simulink model "Final_closeloop_sinus"  (R2024b)
settings: Solver=ode23s  StartTime=0.0  StopTime=150  RelTol=1e-3
libraries: slpidlib x16
(part 1 of 2)
settings Model: Creator=thomasmacbookpro  LastModifiedBy=thomasmacbookpro
settings OptimizationCC: ReuseModelBlockBuffer=off
settings RTWCC: GPUComputeCapability=3.5

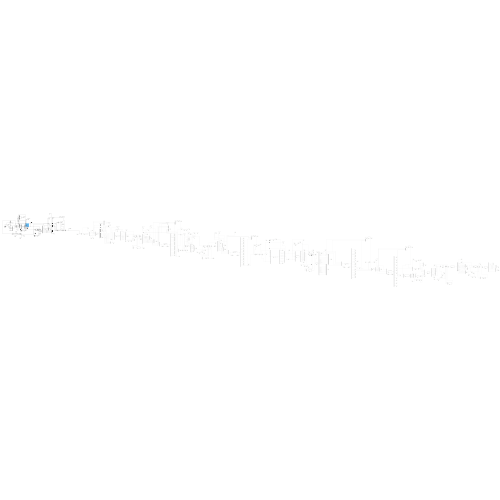
[thumbnail: Simulink's stored preview of the top-level diagram]
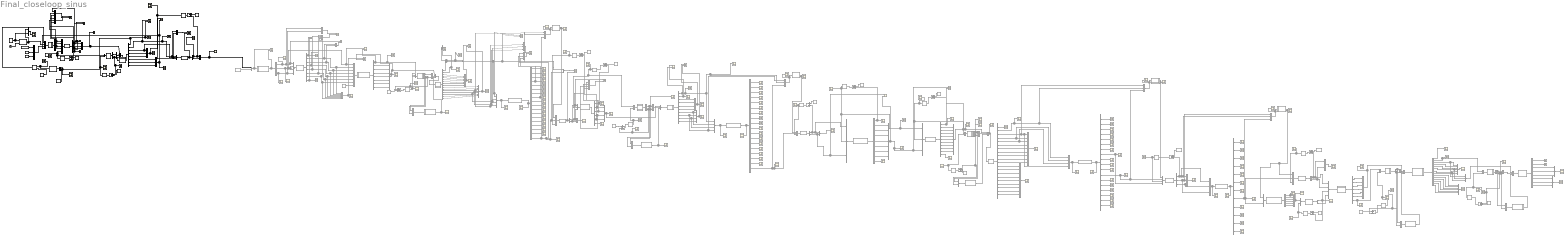
== system Final_closeloop_sinus ==
  " Q, Recycle" : Scope
  % Purge : Constant  Value=0.8
  AC-401:404 : S-Function  Commented=on  FunctionName=AC_Chromatography  Parameters=2  SFunctionDeploymentMode=off  EnableBusSupport=off
  AEX-201:204 : S-Function  Commented=on  FunctionName=AEX_Chromatography  Parameters=2  SFunctionDeploymentMode=off  EnableBusSupport=off
  AEX-301:304 : S-Function  Commented=on  FunctionName=AEX_Chromatography2  Parameters=2  SFunctionDeploymentMode=off  EnableBusSupport=off
  AEX:201:204 C : Scope  Commented=on  NumInputPorts=2
  AEX:201:204,Q IN/OUT1 : Scope  Commented=on  NumInputPorts=2
  "Area, UF-201" : Scope  Commented=on
  "Area, UF-301" : Scope  Commented=on
  "C, Glu, media [g/L]" : Constant  Value=18.1
  "C, N, media [g/L]" : Constant  Value=5.25
  "C, PE, 14" : Scope  Commented=on
  "C, PE, 22" : Scope  Commented=on
  "C, PE-1" : Scope
  "C, PE-2" : Scope  Commented=on
  "C, PE-3" : Scope  Commented=on
  "C, RE, 32" : Scope  Commented=on
  "C, RE, 4" : Scope
  "C, RE-1" : Scope  Commented=on
  "C, RE-2" : Scope  Commented=on
  "C, RE-3" : Scope  Commented=on
  "C, X, media [g/L]" : Constant  Value=0.22
  "C, alkaline lysis, out" : Scope  Commented=on
  "C, mRNA-LNP, PE, 48" : Scope  Commented=on
  "C, neutralization out" : Scope  Commented=on
  "C, output" : Scope  Commented=on
  "C,RE, 47" : Scope  Commented=on
  C,X : Scope  Commented=on
  CH3CO2K [M] : Constant  Commented=on  Value=3
  Clock : Clock
  Constant : Constant  Value=100
  Constant1 : Constant  Value=1.85
  Constant10 : Constant  Commented=on  Value=1.85
  Constant11 : Constant  Commented=on  Value=0.4507
  Constant12 : Constant  Commented=on  Value=0.2845
  Constant13 : Constant  Commented=on  Value=4.827
  Constant14 : Constant  Commented=on  Value=8
  Constant15 : Constant  Commented=on  Value=1.4
  Constant16 : Constant  Value=2.72
  Constant2 : Constant  Value=2.567
  Constant3 : Constant  Commented=on  Value=1.85
  Constant4 : Constant  Commented=on  Value=5.056
  Constant5 : Constant  Commented=on  Value=20
  Constant6 : Constant  Commented=on  Value=1.85
  Constant7 : Constant  Commented=on  Value=2.253
  Constant8 : Constant  Commented=on  Value=20
  Constant9 : Constant  Commented=on  Value=1.13
  Delay block : VariableTransportDelay  VariableDelayType=Variable transport delay  MaximumDelay=10
  Delay time : Constant  Value=0.01
  Demux : Demux  Outputs=5
  Demux1 : Demux  Outputs=8
  Demux10 : Demux  Commented=on  Outputs=18
  Demux{7,11,14,16,20,24..25,27,31} (9 alike) : Demux  Commented=on  Outputs=2
  Demux12 : Demux  Commented=on  Outputs=6
  Demux13 : Demux  Commented=on  Outputs=10
  Demux15 : Demux  Commented=on  Outputs=18
  Demux17 : Demux  Commented=on  Outputs=9
  Demux18 : Demux  Commented=on  Outputs=11
  Demux19 : Demux  Commented=on  Outputs=20
  Demux2 : Demux
  Demux21 : Demux  Commented=on  Outputs=18
  Demux22 : Demux  Commented=on  Outputs=12
  Demux23 : Demux  Commented=on  Outputs=3
  Demux26 : Demux  Commented=on  Outputs=7
  Demux28 : Demux  Commented=on  Outputs=14
  Demux29 : Demux  Commented=on  Outputs=6
  Demux3 : Demux  Outputs=2
  Demux32 : Demux  Commented=on  Outputs=8
  Demux4 : Demux  Outputs=2
  Demux5 : Demux  Commented=on  Outputs=8
  Demux6 : Demux  Commented=on  Outputs=16
  Demux8 : Demux  Commented=on  Outputs=3
  Demux9 : Demux  Commented=on  Outputs=8
  HIC-401:404 : S-Function  Commented=on  FunctionName=HIC_Chromatography  Parameters=2  SFunctionDeploymentMode=off  EnableBusSupport=off
  IVT : Scope  Commented=on
  "Input, AC-401:404" : Scope  Commented=on
  "Input, AEX-201:204" : Scope  Commented=on
  "Input, AEX-301:304" : Scope  Commented=on
  "Intput, HIC-401:404" : Scope  Commented=on
  M-101 : MATLAB Function  TreatAsAtomicUnit=on
  M-501 : S-Function  Commented=on  FunctionName=M_501  SFunctionDeploymentMode=off  EnableBusSupport=off
  MATLAB Function : MATLAB Function  Commented=on  TreatAsAtomicUnit=on
  MATLAB Function1 : MATLAB Function  Commented=on  TreatAsAtomicUnit=on
  MATLAB Function10 : MATLAB Function  Commented=on  TreatAsAtomicUnit=on
  MATLAB Function14 : MATLAB Function  Commented=on  TreatAsAtomicUnit=on
  MATLAB Function15 : MATLAB Function  Commented=on  TreatAsAtomicUnit=on
  MATLAB Function18 : MATLAB Function  Commented=on  TreatAsAtomicUnit=on
  MATLAB Function2 : MATLAB Function  Commented=on  TreatAsAtomicUnit=on
  MATLAB Function3 : MATLAB Function  Commented=on  TreatAsAtomicUnit=on
  MATLAB Function4 : MATLAB Function  Commented=on  TreatAsAtomicUnit=on
  MATLAB Function5 : MATLAB Function  Commented=on  TreatAsAtomicUnit=on
  MATLAB Function6 : MATLAB Function  Commented=on  TreatAsAtomicUnit=on
  MATLAB Function7 : MATLAB Function  Commented=on  TreatAsAtomicUnit=on
  MATLAB Function8 : MATLAB Function  TreatAsAtomicUnit=on
  MF-501 : MATLAB Function  Commented=on  TreatAsAtomicUnit=on
  MM-501 : MATLAB Function  Commented=on  TreatAsAtomicUnit=on
  Mux : Mux
  Mux{1,9..10,13..14,25,71} (7 alike) : Mux  Inputs=3
  Mux{4..6,8,11,21,79} (7 alike) : Mux  Inputs=2
  Mux{3,12,15,22,29,31..32,38,44..45,59,61..62,67..70,74..75,80..81,83,86,91} (24 alike) : Mux  Commented=on  Inputs=2
  Mux{16..17,24,41} (4 alike) : Mux  Commented=on  Inputs=7
  Mux{18,58,60,64,66} (5 alike) : Mux  Commented=on  Inputs=6
  Mux{19..20,26,30,35,39..40,42,47,49,51,56,63,72..73,76,78,84..85,87,89..90} (22 alike) : Mux  Commented=on  Inputs=3
  Mux2 : Mux  Inputs=5
  Mux23 : Mux  Commented=on  Inputs=8
  Mux{7,27,33..34,36..37,50,55,57,82,88} (11 alike) : Mux  Commented=on
  Mux43 : Mux  Commented=on  Inputs=9
  Mux46 : Mux  Commented=on  Inputs=9
  Mux48 : Mux  Commented=on  Inputs=9
  NF-501 : MATLAB Function  Commented=on  TreatAsAtomicUnit=on
  NaOH [M] : Constant  Commented=on  Value=0.42
  "Neutralization, IN/OUT2" : Scope  Commented=on  NumInputPorts=2
  Neutralization,flow IN/OUT1 : Scope  Commented=on  NumInputPorts=2
  "Output, AC-401:404" : Scope  Commented=on
  "Output, AEX-201:204" : Scope  Commented=on
  "Output, AEX-301:304" : Scope  Commented=on
  "Output, HIC-401:404" : Scope  Commented=on
  P : MATLAB Function  TreatAsAtomicUnit=on
  PID Controller : slpidlib/PID Controller  Controller=PI  Form=Parallel  TimeDomain=Continuous-time  UseExternalTs=off  SampleTime=-1  IntegratorMethod=Forward Euler  FilterMethod=Forward Euler  ControllerParametersSource=internal  P=-20  I=-30  UseKiTs=off  D=0  UseExternalDerivativeSource=off  N=100  UseFilter=on  TunerSelectOption=Transfer Function Based (PID Tuner App)  InitialConditionSource=internal  InitialConditionForIntegrator=3.33  InitialConditionForFilter=0  DifferentiatorICPrevScaledInput=0  ExternalReset=none  TrackingMode=off  Kt=1  LimitOutput=on  SatLimitsSource=internal  UpperSaturationLimit=inf  LowerSaturationLimit=-inf  LinearizeAsGain=on  AntiWindupMode=clamping  Kb=1  LimitIntegrator=off  UpperIntegratorSaturationLimit=inf  LowerIntegratorSaturationLimit=-inf  POutMin=[]  POutMax=[]  IOutMin=[]  IOutMax=[]  DOutMin=[]  DOutMax=[]  NOutMin=[]  NOutMax=[]  SumOutMin=[]  SumOutMax=[]  SaturationOutMin=[]  SaturationOutMax=[]  PParamMin=[]  PParamMax=[]  IParamMin=[]  IParamMax=[]  DParamMin=[]  DParamMax=[]  NParamMin=[]  NParamMax=[]  KbParamMin=[]  KbParamMax=[]  KtParamMin=[]  KtParamMax=[]  KbOutMin=[]  KbOutMax=[]  KtOutMin=[]  KtOutMax=[]  IntegratorOutMin=[]  IntegratorOutMax=[]  FilterOutMin=[]  FilterOutMax=[]  SumI1OutMin=[]  SumI1OutMax=[]  SumI2OutMin=[]  SumI2OutMax=[]  SumI3OutMin=[]  SumI3OutMax=[]  SumI4OutMin=[]  SumI4OutMax=[]  SumDOutMin=[]  SumDOutMax=[]  DifferentiatorOutMin=[]  DifferentiatorOutMax=[]  FilterDiffOutCoefMin=[]  FilterDiffOutCoefMax=[]  ReciprocalOutMin=[]  ReciprocalOutMax=[]  SumDenOutMin=[]  SumDenOutMax=[]  SumNumOutMin=[]  SumNumOutMax=[]  DivideOutMin=[]  DivideOutMax=[]  UdiffTsProdOutMin=[]  UdiffTsProdOutMax=[]  NTsProdOutMin=[]  NTsProdOutMax=[]  UintegralTsProdOutMin=[]  UintegralTsProdOutMax=[]  UngainTsProdOutMin=[]  UngainTsProdOutMax=[]  ClampingZeroOutDataTypeStr=Inherit: Inherit via back propagation  ClampingZeroOutMin=[]  ClampingZeroOutMax=[]  FilterDenConstantOutDataTypeStr=Inherit: Inherit via back propagation  FilterDenConstantOutMin=[]  FilterDenConstantOutMax=[]  PCopyOutDataTypeStr=Inherit: Inherit via back propagation  PCopyOutMin=[]  PCopyOutMax=[]  NCopyOutDataTypeStr=Inherit: Inherit via back propagation  NCopyOutMin=[]  NCopyOutMax=[]  IntegratorContinuousStateAttributes=''  IntegratorStateMustResolveToSignalObject=off  IntegratorRTWStateStorageClass=Auto  FilterContinuousStateAttributes=''  FilterStateMustResolveToSignalObject=off  FilterRTWStateStorageClass=Auto  ParallelPVariant=InternalParameters  IdealPVariant=Disabled  IVariant=InternalParameters  DVariant=Disabled  IntegratorVariant=Continuous  SatVariant=Enabled  AWVariant=ContClampingParallel  PCopyVariant=Disabled  TRVariant=Disabled  FdbkBlocksVariant=Forward  IdealPFdbkVariant=Disabled  SatFdbkVariant=Disabled  DerivativeFilterVariant=Disabled  NVariant=Disabled  NCopyVariant=Disabled_SignalSpec  FilterICVariant=Disabled  IntegratorICVariant=InternalICs  ExternalResetVariant=Disabled  TRSumVariant=Passthrough  SumFdbkVariant=Disabled  SumVariant=Sum_PI  TsampFilterVariant=InternalTs  TsampNgainVariant=Passthrough  TsampIntegralVariant=Disabled_SignalSpec  ExternalSaturationOutDataTypeStr=Inherit: Same as second input  DerivativeSourceVariant=Disabled  PreIntVariant=InternalPreInt
  PID Controller1 : slpidlib/PID Controller  Controller=PI  Form=Parallel  TimeDomain=Continuous-time  UseExternalTs=off  SampleTime=-1  IntegratorMethod=Forward Euler  FilterMethod=Forward Euler  ControllerParametersSource=internal  P=100  I=1762.06127367321  UseKiTs=off  D=0  UseExternalDerivativeSource=off  N=100  UseFilter=on  TunerSelectOption=Transfer Function Based (PID Tuner App)  InitialConditionSource=internal  InitialConditionForIntegrator=1134  InitialConditionForFilter=0  DifferentiatorICPrevScaledInput=0  ExternalReset=none  TrackingMode=off  Kt=1  LimitOutput=on  SatLimitsSource=internal  UpperSaturationLimit=inf  LowerSaturationLimit=-inf  LinearizeAsGain=on  AntiWindupMode=none  Kb=1  LimitIntegrator=off  UpperIntegratorSaturationLimit=inf  LowerIntegratorSaturationLimit=-inf  POutMin=[]  POutMax=[]  IOutMin=[]  IOutMax=[]  DOutMin=[]  DOutMax=[]  NOutMin=[]  NOutMax=[]  SumOutMin=[]  SumOutMax=[]  SaturationOutMin=[]  SaturationOutMax=[]  PParamMin=[]  PParamMax=[]  IParamMin=[]  IParamMax=[]  DParamMin=[]  DParamMax=[]  NParamMin=[]  NParamMax=[]  KbParamMin=[]  KbParamMax=[]  KtParamMin=[]  KtParamMax=[]  KbOutMin=[]  KbOutMax=[]  KtOutMin=[]  KtOutMax=[]  IntegratorOutMin=[]  IntegratorOutMax=[]  FilterOutMin=[]  FilterOutMax=[]  SumI1OutMin=[]  SumI1OutMax=[]  SumI2OutMin=[]  SumI2OutMax=[]  SumI3OutMin=[]  SumI3OutMax=[]  SumI4OutMin=[]  SumI4OutMax=[]  SumDOutMin=[]  SumDOutMax=[]  DifferentiatorOutMin=[]  DifferentiatorOutMax=[]  FilterDiffOutCoefMin=[]  FilterDiffOutCoefMax=[]  ReciprocalOutMin=[]  ReciprocalOutMax=[]  SumDenOutMin=[]  SumDenOutMax=[]  SumNumOutMin=[]  SumNumOutMax=[]  DivideOutMin=[]  DivideOutMax=[]  UdiffTsProdOutMin=[]  UdiffTsProdOutMax=[]  NTsProdOutMin=[]  NTsProdOutMax=[]  UintegralTsProdOutMin=[]  UintegralTsProdOutMax=[]  UngainTsProdOutMin=[]  UngainTsProdOutMax=[]  ClampingZeroOutDataTypeStr=Inherit: Inherit via back propagation  ClampingZeroOutMin=[]  ClampingZeroOutMax=[]  FilterDenConstantOutDataTypeStr=Inherit: Inherit via back propagation  FilterDenConstantOutMin=[]  FilterDenConstantOutMax=[]  PCopyOutDataTypeStr=Inherit: Inherit via back propagation  PCopyOutMin=[]  PCopyOutMax=[]  NCopyOutDataTypeStr=Inherit: Inherit via back propagation  NCopyOutMin=[]  NCopyOutMax=[]  IntegratorContinuousStateAttributes=''  IntegratorStateMustResolveToSignalObject=off  IntegratorRTWStateStorageClass=Auto  FilterContinuousStateAttributes=''  FilterStateMustResolveToSignalObject=off  FilterRTWStateStorageClass=Auto  ParallelPVariant=InternalParameters  IdealPVariant=Disabled  IVariant=InternalParameters  DVariant=Disabled  IntegratorVariant=Continuous  SatVariant=Enabled  AWVariant=Passthrough  PCopyVariant=Disabled  TRVariant=Disabled  FdbkBlocksVariant=Forward  IdealPFdbkVariant=Disabled  SatFdbkVariant=Disabled  DerivativeFilterVariant=Disabled  NVariant=Disabled  NCopyVariant=Disabled_SignalSpec  FilterICVariant=Disabled  IntegratorICVariant=InternalICs  ExternalResetVariant=Disabled  TRSumVariant=Passthrough  SumFdbkVariant=Disabled  SumVariant=Sum_PI  TsampFilterVariant=InternalTs  TsampNgainVariant=Passthrough  TsampIntegralVariant=Disabled_SignalSpec  ExternalSaturationOutDataTypeStr=Inherit: Same as second input  DerivativeSourceVariant=Disabled  PreIntVariant=InternalPreInt
  PID Controller10 : slpidlib/PID Controller  Commented=on  Controller=PI  Form=Parallel  TimeDomain=Continuous-time  UseExternalTs=off  SampleTime=-1  IntegratorMethod=Forward Euler  FilterMethod=Forward Euler  ControllerParametersSource=internal  P=0  I=1695.13781714754  UseKiTs=off  D=0  UseExternalDerivativeSource=off  N=100  UseFilter=on  TunerSelectOption=Transfer Function Based (PID Tuner App)  InitialConditionSource=internal  InitialConditionForIntegrator=1118  InitialConditionForFilter=0  DifferentiatorICPrevScaledInput=0  ExternalReset=none  TrackingMode=off  Kt=1  LimitOutput=off  SatLimitsSource=internal  UpperSaturationLimit=inf  LowerSaturationLimit=-inf  LinearizeAsGain=on  AntiWindupMode=none  Kb=1  LimitIntegrator=off  UpperIntegratorSaturationLimit=inf  LowerIntegratorSaturationLimit=-inf  POutMin=[]  POutMax=[]  IOutMin=[]  IOutMax=[]  DOutMin=[]  DOutMax=[]  NOutMin=[]  NOutMax=[]  SumOutMin=[]  SumOutMax=[]  SaturationOutMin=[]  SaturationOutMax=[]  PParamMin=[]  PParamMax=[]  IParamMin=[]  IParamMax=[]  DParamMin=[]  DParamMax=[]  NParamMin=[]  NParamMax=[]  KbParamMin=[]  KbParamMax=[]  KtParamMin=[]  KtParamMax=[]  KbOutMin=[]  KbOutMax=[]  KtOutMin=[]  KtOutMax=[]  IntegratorOutMin=[]  IntegratorOutMax=[]  FilterOutMin=[]  FilterOutMax=[]  SumI1OutMin=[]  SumI1OutMax=[]  SumI2OutMin=[]  SumI2OutMax=[]  SumI3OutMin=[]  SumI3OutMax=[]  SumI4OutMin=[]  SumI4OutMax=[]  SumDOutMin=[]  SumDOutMax=[]  DifferentiatorOutMin=[]  DifferentiatorOutMax=[]  FilterDiffOutCoefMin=[]  FilterDiffOutCoefMax=[]  ReciprocalOutMin=[]  ReciprocalOutMax=[]  SumDenOutMin=[]  SumDenOutMax=[]  SumNumOutMin=[]  SumNumOutMax=[]  DivideOutMin=[]  DivideOutMax=[]  UdiffTsProdOutMin=[]  UdiffTsProdOutMax=[]  NTsProdOutMin=[]  NTsProdOutMax=[]  UintegralTsProdOutMin=[]  UintegralTsProdOutMax=[]  UngainTsProdOutMin=[]  UngainTsProdOutMax=[]  ClampingZeroOutDataTypeStr=Inherit: Inherit via back propagation  ClampingZeroOutMin=[]  ClampingZeroOutMax=[]  FilterDenConstantOutDataTypeStr=Inherit: Inherit via back propagation  FilterDenConstantOutMin=[]  FilterDenConstantOutMax=[]  PCopyOutDataTypeStr=Inherit: Inherit via back propagation  PCopyOutMin=[]  PCopyOutMax=[]  NCopyOutDataTypeStr=Inherit: Inherit via back propagation  NCopyOutMin=[]  NCopyOutMax=[]  IntegratorContinuousStateAttributes=''  IntegratorStateMustResolveToSignalObject=off  IntegratorRTWStateStorageClass=Auto  FilterContinuousStateAttributes=''  FilterStateMustResolveToSignalObject=off  FilterRTWStateStorageClass=Auto  ParallelPVariant=InternalParameters  IdealPVariant=Disabled  IVariant=InternalParameters  DVariant=Disabled  IntegratorVariant=Continuous  SatVariant=Disabled  AWVariant=Passthrough  PCopyVariant=Disabled  TRVariant=Disabled  FdbkBlocksVariant=Forward  IdealPFdbkVariant=Disabled  SatFdbkVariant=Disabled  DerivativeFilterVariant=Disabled  NVariant=Disabled  NCopyVariant=Disabled_SignalSpec  FilterICVariant=Disabled  IntegratorICVariant=InternalICs  ExternalResetVariant=Disabled  TRSumVariant=Passthrough  SumFdbkVariant=Disabled  SumVariant=Sum_PI  TsampFilterVariant=InternalTs  TsampNgainVariant=Passthrough  TsampIntegralVariant=Disabled_SignalSpec  ExternalSaturationOutDataTypeStr=Inherit: Same as second input  DerivativeSourceVariant=Disabled  PreIntVariant=InternalPreInt
  PID Controller11 : slpidlib/PID Controller  Commented=on  Controller=PI  Form=Parallel  TimeDomain=Continuous-time  UseExternalTs=off  SampleTime=-1  IntegratorMethod=Forward Euler  FilterMethod=Forward Euler  ControllerParametersSource=internal  P=-6.6059228190806  I=-0.763863716153279  UseKiTs=off  D=0  UseExternalDerivativeSource=off  N=100  UseFilter=on  TunerSelectOption=Transfer Function Based (PID Tuner App)  InitialConditionSource=internal  InitialConditionForIntegrator=0.4507  InitialConditionForFilter=0  DifferentiatorICPrevScaledInput=0  ExternalReset=none  TrackingMode=off  Kt=1  LimitOutput=off  SatLimitsSource=internal  UpperSaturationLimit=inf  LowerSaturationLimit=-inf  LinearizeAsGain=on  AntiWindupMode=none  Kb=1  LimitIntegrator=off  UpperIntegratorSaturationLimit=inf  LowerIntegratorSaturationLimit=-inf  POutMin=[]  POutMax=[]  IOutMin=[]  IOutMax=[]  DOutMin=[]  DOutMax=[]  NOutMin=[]  NOutMax=[]  SumOutMin=[]  SumOutMax=[]  SaturationOutMin=[]  SaturationOutMax=[]  PParamMin=[]  PParamMax=[]  IParamMin=[]  IParamMax=[]  DParamMin=[]  DParamMax=[]  NParamMin=[]  NParamMax=[]  KbParamMin=[]  KbParamMax=[]  KtParamMin=[]  KtParamMax=[]  KbOutMin=[]  KbOutMax=[]  KtOutMin=[]  KtOutMax=[]  IntegratorOutMin=[]  IntegratorOutMax=[]  FilterOutMin=[]  FilterOutMax=[]  SumI1OutMin=[]  SumI1OutMax=[]  SumI2OutMin=[]  SumI2OutMax=[]  SumI3OutMin=[]  SumI3OutMax=[]  SumI4OutMin=[]  SumI4OutMax=[]  SumDOutMin=[]  SumDOutMax=[]  DifferentiatorOutMin=[]  DifferentiatorOutMax=[]  FilterDiffOutCoefMin=[]  FilterDiffOutCoefMax=[]  ReciprocalOutMin=[]  ReciprocalOutMax=[]  SumDenOutMin=[]  SumDenOutMax=[]  SumNumOutMin=[]  SumNumOutMax=[]  DivideOutMin=[]  DivideOutMax=[]  UdiffTsProdOutMin=[]  UdiffTsProdOutMax=[]  NTsProdOutMin=[]  NTsProdOutMax=[]  UintegralTsProdOutMin=[]  UintegralTsProdOutMax=[]  UngainTsProdOutMin=[]  UngainTsProdOutMax=[]  ClampingZeroOutDataTypeStr=Inherit: Inherit via back propagation  ClampingZeroOutMin=[]  ClampingZeroOutMax=[]  FilterDenConstantOutDataTypeStr=Inherit: Inherit via back propagation  FilterDenConstantOutMin=[]  FilterDenConstantOutMax=[]  PCopyOutDataTypeStr=Inherit: Inherit via back propagation  PCopyOutMin=[]  PCopyOutMax=[]  NCopyOutDataTypeStr=Inherit: Inherit via back propagation  NCopyOutMin=[]  NCopyOutMax=[]  IntegratorContinuousStateAttributes=''  IntegratorStateMustResolveToSignalObject=off  IntegratorRTWStateStorageClass=Auto  FilterContinuousStateAttributes=''  FilterStateMustResolveToSignalObject=off  FilterRTWStateStorageClass=Auto  ParallelPVariant=InternalParameters  IdealPVariant=Disabled  IVariant=InternalParameters  DVariant=Disabled  IntegratorVariant=Continuous  SatVariant=Disabled  AWVariant=Passthrough  PCopyVariant=Disabled  TRVariant=Disabled  FdbkBlocksVariant=Forward  IdealPFdbkVariant=Disabled  SatFdbkVariant=Disabled  DerivativeFilterVariant=Disabled  NVariant=Disabled  NCopyVariant=Disabled_SignalSpec  FilterICVariant=Disabled  IntegratorICVariant=InternalICs  ExternalResetVariant=Disabled  TRSumVariant=Passthrough  SumFdbkVariant=Disabled  SumVariant=Sum_PI  TsampFilterVariant=InternalTs  TsampNgainVariant=Passthrough  TsampIntegralVariant=Disabled_SignalSpec  ExternalSaturationOutDataTypeStr=Inherit: Same as second input  DerivativeSourceVariant=Disabled  PreIntVariant=InternalPreInt
  PID Controller12 : slpidlib/PID Controller  Commented=on  Controller=PI  Form=Parallel  TimeDomain=Continuous-time  UseExternalTs=off  SampleTime=-1  IntegratorMethod=Forward Euler  FilterMethod=Forward Euler  ControllerParametersSource=internal  P=-6.9172503700087  I=-0.837559909578323  UseKiTs=off  D=0  UseExternalDerivativeSource=off  N=100  UseFilter=on  TunerSelectOption=Transfer Function Based (PID Tuner App)  InitialConditionSource=internal  InitialConditionForIntegrator=0.2845  InitialConditionForFilter=0  DifferentiatorICPrevScaledInput=0  ExternalReset=none  TrackingMode=off  Kt=1  LimitOutput=off  SatLimitsSource=internal  UpperSaturationLimit=inf  LowerSaturationLimit=-inf  LinearizeAsGain=on  AntiWindupMode=none  Kb=1  LimitIntegrator=off  UpperIntegratorSaturationLimit=inf  LowerIntegratorSaturationLimit=-inf  POutMin=[]  POutMax=[]  IOutMin=[]  IOutMax=[]  DOutMin=[]  DOutMax=[]  NOutMin=[]  NOutMax=[]  SumOutMin=[]  SumOutMax=[]  SaturationOutMin=[]  SaturationOutMax=[]  PParamMin=[]  PParamMax=[]  IParamMin=[]  IParamMax=[]  DParamMin=[]  DParamMax=[]  NParamMin=[]  NParamMax=[]  KbParamMin=[]  KbParamMax=[]  KtParamMin=[]  KtParamMax=[]  KbOutMin=[]  KbOutMax=[]  KtOutMin=[]  KtOutMax=[]  IntegratorOutMin=[]  IntegratorOutMax=[]  FilterOutMin=[]  FilterOutMax=[]  SumI1OutMin=[]  SumI1OutMax=[]  SumI2OutMin=[]  SumI2OutMax=[]  SumI3OutMin=[]  SumI3OutMax=[]  SumI4OutMin=[]  SumI4OutMax=[]  SumDOutMin=[]  SumDOutMax=[]  DifferentiatorOutMin=[]  DifferentiatorOutMax=[]  FilterDiffOutCoefMin=[]  FilterDiffOutCoefMax=[]  ReciprocalOutMin=[]  ReciprocalOutMax=[]  SumDenOutMin=[]  SumDenOutMax=[]  SumNumOutMin=[]  SumNumOutMax=[]  DivideOutMin=[]  DivideOutMax=[]  UdiffTsProdOutMin=[]  UdiffTsProdOutMax=[]  NTsProdOutMin=[]  NTsProdOutMax=[]  UintegralTsProdOutMin=[]  UintegralTsProdOutMax=[]  UngainTsProdOutMin=[]  UngainTsProdOutMax=[]  ClampingZeroOutDataTypeStr=Inherit: Inherit via back propagation  ClampingZeroOutMin=[]  ClampingZeroOutMax=[]  FilterDenConstantOutDataTypeStr=Inherit: Inherit via back propagation  FilterDenConstantOutMin=[]  FilterDenConstantOutMax=[]  PCopyOutDataTypeStr=Inherit: Inherit via back propagation  PCopyOutMin=[]  PCopyOutMax=[]  NCopyOutDataTypeStr=Inherit: Inherit via back propagation  NCopyOutMin=[]  NCopyOutMax=[]  IntegratorContinuousStateAttributes=''  IntegratorStateMustResolveToSignalObject=off  IntegratorRTWStateStorageClass=Auto  FilterContinuousStateAttributes=''  FilterStateMustResolveToSignalObject=off  FilterRTWStateStorageClass=Auto  ParallelPVariant=InternalParameters  IdealPVariant=Disabled  IVariant=InternalParameters  DVariant=Disabled  IntegratorVariant=Continuous  SatVariant=Disabled  AWVariant=Passthrough  PCopyVariant=Disabled  TRVariant=Disabled  FdbkBlocksVariant=Forward  IdealPFdbkVariant=Disabled  SatFdbkVariant=Disabled  DerivativeFilterVariant=Disabled  NVariant=Disabled  NCopyVariant=Disabled_SignalSpec  FilterICVariant=Disabled  IntegratorICVariant=InternalICs  ExternalResetVariant=Disabled  TRSumVariant=Passthrough  SumFdbkVariant=Disabled  SumVariant=Sum_PI  TsampFilterVariant=InternalTs  TsampNgainVariant=Passthrough  TsampIntegralVariant=Disabled_SignalSpec  ExternalSaturationOutDataTypeStr=Inherit: Same as second input  DerivativeSourceVariant=Disabled  PreIntVariant=InternalPreInt
  PID Controller13 : slpidlib/PID Controller  Commented=on  Controller=PI  Form=Parallel  TimeDomain=Continuous-time  UseExternalTs=off  SampleTime=-1  IntegratorMethod=Forward Euler  FilterMethod=Forward Euler  ControllerParametersSource=internal  P=-6.91725036983727  I=-0.837559909557566  UseKiTs=off  D=0  UseExternalDerivativeSource=off  N=100  UseFilter=on  TunerSelectOption=Transfer Function Based (PID Tuner App)  InitialConditionSource=internal  InitialConditionForIntegrator=4  InitialConditionForFilter=0  DifferentiatorICPrevScaledInput=0  ExternalReset=none  TrackingMode=off  Kt=1  LimitOutput=off  SatLimitsSource=internal  UpperSaturationLimit=inf  LowerSaturationLimit=-inf  LinearizeAsGain=on  AntiWindupMode=none  Kb=1  LimitIntegrator=off  UpperIntegratorSaturationLimit=inf  LowerIntegratorSaturationLimit=-inf  POutMin=[]  POutMax=[]  IOutMin=[]  IOutMax=[]  DOutMin=[]  DOutMax=[]  NOutMin=[]  NOutMax=[]  SumOutMin=[]  SumOutMax=[]  SaturationOutMin=[]  SaturationOutMax=[]  PParamMin=[]  PParamMax=[]  IParamMin=[]  IParamMax=[]  DParamMin=[]  DParamMax=[]  NParamMin=[]  NParamMax=[]  KbParamMin=[]  KbParamMax=[]  KtParamMin=[]  KtParamMax=[]  KbOutMin=[]  KbOutMax=[]  KtOutMin=[]  KtOutMax=[]  IntegratorOutMin=[]  IntegratorOutMax=[]  FilterOutMin=[]  FilterOutMax=[]  SumI1OutMin=[]  SumI1OutMax=[]  SumI2OutMin=[]  SumI2OutMax=[]  SumI3OutMin=[]  SumI3OutMax=[]  SumI4OutMin=[]  SumI4OutMax=[]  SumDOutMin=[]  SumDOutMax=[]  DifferentiatorOutMin=[]  DifferentiatorOutMax=[]  FilterDiffOutCoefMin=[]  FilterDiffOutCoefMax=[]  ReciprocalOutMin=[]  ReciprocalOutMax=[]  SumDenOutMin=[]  SumDenOutMax=[]  SumNumOutMin=[]  SumNumOutMax=[]  DivideOutMin=[]  DivideOutMax=[]  UdiffTsProdOutMin=[]  UdiffTsProdOutMax=[]  NTsProdOutMin=[]  NTsProdOutMax=[]  UintegralTsProdOutMin=[]  UintegralTsProdOutMax=[]  UngainTsProdOutMin=[]  UngainTsProdOutMax=[]  ClampingZeroOutDataTypeStr=Inherit: Inherit via back propagation  ClampingZeroOutMin=[]  ClampingZeroOutMax=[]  FilterDenConstantOutDataTypeStr=Inherit: Inherit via back propagation  FilterDenConstantOutMin=[]  FilterDenConstantOutMax=[]  PCopyOutDataTypeStr=Inherit: Inherit via back propagation  PCopyOutMin=[]  PCopyOutMax=[]  NCopyOutDataTypeStr=Inherit: Inherit via back propagation  NCopyOutMin=[]  NCopyOutMax=[]  IntegratorContinuousStateAttributes=''  IntegratorStateMustResolveToSignalObject=off  IntegratorRTWStateStorageClass=Auto  FilterContinuousStateAttributes=''  FilterStateMustResolveToSignalObject=off  FilterRTWStateStorageClass=Auto  ParallelPVariant=InternalParameters  IdealPVariant=Disabled  IVariant=InternalParameters  DVariant=Disabled  IntegratorVariant=Continuous  SatVariant=Disabled  AWVariant=Passthrough  PCopyVariant=Disabled  TRVariant=Disabled  FdbkBlocksVariant=Forward  IdealPFdbkVariant=Disabled  SatFdbkVariant=Disabled  DerivativeFilterVariant=Disabled  NVariant=Disabled  NCopyVariant=Disabled_SignalSpec  FilterICVariant=Disabled  IntegratorICVariant=InternalICs  ExternalResetVariant=Disabled  TRSumVariant=Passthrough  SumFdbkVariant=Disabled  SumVariant=Sum_PI  TsampFilterVariant=InternalTs  TsampNgainVariant=Passthrough  TsampIntegralVariant=Disabled_SignalSpec  ExternalSaturationOutDataTypeStr=Inherit: Same as second input  DerivativeSourceVariant=Disabled  PreIntVariant=InternalPreInt
  PID Controller14 : slpidlib/PID Controller  Commented=on  Controller=PI  Form=Parallel  TimeDomain=Continuous-time  UseExternalTs=off  SampleTime=-1  IntegratorMethod=Forward Euler  FilterMethod=Forward Euler  ControllerParametersSource=internal  P=0  I=1138.66901210131  UseKiTs=off  D=0  UseExternalDerivativeSource=off  N=100  UseFilter=on  TunerSelectOption=Transfer Function Based (PID Tuner App)  InitialConditionSource=internal  InitialConditionForIntegrator=2334  InitialConditionForFilter=0  DifferentiatorICPrevScaledInput=0  ExternalReset=none  TrackingMode=off  Kt=1  LimitOutput=off  SatLimitsSource=internal  UpperSaturationLimit=inf  LowerSaturationLimit=-inf  LinearizeAsGain=on  AntiWindupMode=none  Kb=1  LimitIntegrator=off  UpperIntegratorSaturationLimit=inf  LowerIntegratorSaturationLimit=-inf  POutMin=[]  POutMax=[]  IOutMin=[]  IOutMax=[]  DOutMin=[]  DOutMax=[]  NOutMin=[]  NOutMax=[]  SumOutMin=[]  SumOutMax=[]  SaturationOutMin=[]  SaturationOutMax=[]  PParamMin=[]  PParamMax=[]  IParamMin=[]  IParamMax=[]  DParamMin=[]  DParamMax=[]  NParamMin=[]  NParamMax=[]  KbParamMin=[]  KbParamMax=[]  KtParamMin=[]  KtParamMax=[]  KbOutMin=[]  KbOutMax=[]  KtOutMin=[]  KtOutMax=[]  IntegratorOutMin=[]  IntegratorOutMax=[]  FilterOutMin=[]  FilterOutMax=[]  SumI1OutMin=[]  SumI1OutMax=[]  SumI2OutMin=[]  SumI2OutMax=[]  SumI3OutMin=[]  SumI3OutMax=[]  SumI4OutMin=[]  SumI4OutMax=[]  SumDOutMin=[]  SumDOutMax=[]  DifferentiatorOutMin=[]  DifferentiatorOutMax=[]  FilterDiffOutCoefMin=[]  FilterDiffOutCoefMax=[]  ReciprocalOutMin=[]  ReciprocalOutMax=[]  SumDenOutMin=[]  SumDenOutMax=[]  SumNumOutMin=[]  SumNumOutMax=[]  DivideOutMin=[]  DivideOutMax=[]  UdiffTsProdOutMin=[]  UdiffTsProdOutMax=[]  NTsProdOutMin=[]  NTsProdOutMax=[]  UintegralTsProdOutMin=[]  UintegralTsProdOutMax=[]  UngainTsProdOutMin=[]  UngainTsProdOutMax=[]  ClampingZeroOutDataTypeStr=Inherit: Inherit via back propagation  ClampingZeroOutMin=[]  ClampingZeroOutMax=[]  FilterDenConstantOutDataTypeStr=Inherit: Inherit via back propagation  FilterDenConstantOutMin=[]  FilterDenConstantOutMax=[]  PCopyOutDataTypeStr=Inherit: Inherit via back propagation  PCopyOutMin=[]  PCopyOutMax=[]  NCopyOutDataTypeStr=Inherit: Inherit via back propagation  NCopyOutMin=[]  NCopyOutMax=[]  IntegratorContinuousStateAttributes=''  IntegratorStateMustResolveToSignalObject=off  IntegratorRTWStateStorageClass=Auto  FilterContinuousStateAttributes=''  FilterStateMustResolveToSignalObject=off  FilterRTWStateStorageClass=Auto  ParallelPVariant=InternalParameters  IdealPVariant=Disabled  IVariant=InternalParameters  DVariant=Disabled  IntegratorVariant=Continuous  SatVariant=Disabled  AWVariant=Passthrough  PCopyVariant=Disabled  TRVariant=Disabled  FdbkBlocksVariant=Forward  IdealPFdbkVariant=Disabled  SatFdbkVariant=Disabled  DerivativeFilterVariant=Disabled  NVariant=Disabled  NCopyVariant=Disabled_SignalSpec  FilterICVariant=Disabled  IntegratorICVariant=InternalICs  ExternalResetVariant=Disabled  TRSumVariant=Passthrough  SumFdbkVariant=Disabled  SumVariant=Sum_PI  TsampFilterVariant=InternalTs  TsampNgainVariant=Passthrough  TsampIntegralVariant=Disabled_SignalSpec  ExternalSaturationOutDataTypeStr=Inherit: Same as second input  DerivativeSourceVariant=Disabled  PreIntVariant=InternalPreInt
  PID Controller15 : slpidlib/PID Controller  Commented=on  Controller=PI  Form=Parallel  TimeDomain=Continuous-time  UseExternalTs=off  SampleTime=-1  IntegratorMethod=Forward Euler  FilterMethod=Forward Euler  ControllerParametersSource=internal  P=0  I=2710.16235928108  UseKiTs=off  D=0  UseExternalDerivativeSource=off  N=100  UseFilter=on  TunerSelectOption=Transfer Function Based (PID Tuner App)  InitialConditionSource=internal  InitialConditionForIntegrator=964.3  InitialConditionForFilter=0  DifferentiatorICPrevScaledInput=0  ExternalReset=none  TrackingMode=off  Kt=1  LimitOutput=off  SatLimitsSource=internal  UpperSaturationLimit=inf  LowerSaturationLimit=-inf  LinearizeAsGain=on  AntiWindupMode=none  Kb=1  LimitIntegrator=off  UpperIntegratorSaturationLimit=inf  LowerIntegratorSaturationLimit=-inf  POutMin=[]  POutMax=[]  IOutMin=[]  IOutMax=[]  DOutMin=[]  DOutMax=[]  NOutMin=[]  NOutMax=[]  SumOutMin=[]  SumOutMax=[]  SaturationOutMin=[]  SaturationOutMax=[]  PParamMin=[]  PParamMax=[]  IParamMin=[]  IParamMax=[]  DParamMin=[]  DParamMax=[]  NParamMin=[]  NParamMax=[]  KbParamMin=[]  KbParamMax=[]  KtParamMin=[]  KtParamMax=[]  KbOutMin=[]  KbOutMax=[]  KtOutMin=[]  KtOutMax=[]  IntegratorOutMin=[]  IntegratorOutMax=[]  FilterOutMin=[]  FilterOutMax=[]  SumI1OutMin=[]  SumI1OutMax=[]  SumI2OutMin=[]  SumI2OutMax=[]  SumI3OutMin=[]  SumI3OutMax=[]  SumI4OutMin=[]  SumI4OutMax=[]  SumDOutMin=[]  SumDOutMax=[]  DifferentiatorOutMin=[]  DifferentiatorOutMax=[]  FilterDiffOutCoefMin=[]  FilterDiffOutCoefMax=[]  ReciprocalOutMin=[]  ReciprocalOutMax=[]  SumDenOutMin=[]  SumDenOutMax=[]  SumNumOutMin=[]  SumNumOutMax=[]  DivideOutMin=[]  DivideOutMax=[]  UdiffTsProdOutMin=[]  UdiffTsProdOutMax=[]  NTsProdOutMin=[]  NTsProdOutMax=[]  UintegralTsProdOutMin=[]  UintegralTsProdOutMax=[]  UngainTsProdOutMin=[]  UngainTsProdOutMax=[]  ClampingZeroOutDataTypeStr=Inherit: Inherit via back propagation  ClampingZeroOutMin=[]  ClampingZeroOutMax=[]  FilterDenConstantOutDataTypeStr=Inherit: Inherit via back propagation  FilterDenConstantOutMin=[]  FilterDenConstantOutMax=[]  PCopyOutDataTypeStr=Inherit: Inherit via back propagation  PCopyOutMin=[]  PCopyOutMax=[]  NCopyOutDataTypeStr=Inherit: Inherit via back propagation  NCopyOutMin=[]  NCopyOutMax=[]  IntegratorContinuousStateAttributes=''  IntegratorStateMustResolveToSignalObject=off  IntegratorRTWStateStorageClass=Auto  FilterContinuousStateAttributes=''  FilterStateMustResolveToSignalObject=off  FilterRTWStateStorageClass=Auto  ParallelPVariant=InternalParameters  IdealPVariant=Disabled  IVariant=InternalParameters  DVariant=Disabled  IntegratorVariant=Continuous  SatVariant=Disabled  AWVariant=Passthrough  PCopyVariant=Disabled  TRVariant=Disabled  FdbkBlocksVariant=Forward  IdealPFdbkVariant=Disabled  SatFdbkVariant=Disabled  DerivativeFilterVariant=Disabled  NVariant=Disabled  NCopyVariant=Disabled_SignalSpec  FilterICVariant=Disabled  IntegratorICVariant=InternalICs  ExternalResetVariant=Disabled  TRSumVariant=Passthrough  SumFdbkVariant=Disabled  SumVariant=Sum_PI  TsampFilterVariant=InternalTs  TsampNgainVariant=Passthrough  TsampIntegralVariant=Disabled_SignalSpec  ExternalSaturationOutDataTypeStr=Inherit: Same as second input  DerivativeSourceVariant=Disabled  PreIntVariant=InternalPreInt
  PID Controller2 : slpidlib/PID Controller  Controller=PI  Form=Parallel  TimeDomain=Continuous-time  UseExternalTs=off  SampleTime=-1  IntegratorMethod=Forward Euler  FilterMethod=Forward Euler  ControllerParametersSource=internal  P=-7.18723566147925  I=-6.57758159914682  UseKiTs=off  D=0  UseExternalDerivativeSource=off  N=100  UseFilter=on  TunerSelectOption=Transfer Function Based (PID Tuner App)  InitialConditionSource=internal  InitialConditionForIntegrator=0  InitialConditionForFilter=0  DifferentiatorICPrevScaledInput=0  ExternalReset=none  TrackingMode=off  Kt=1  LimitOutput=off  SatLimitsSource=internal  UpperSaturationLimit=inf  LowerSaturationLimit=-inf  LinearizeAsGain=on  AntiWindupMode=none  Kb=1  LimitIntegrator=off  UpperIntegratorSaturationLimit=inf  LowerIntegratorSaturationLimit=-inf  POutMin=[]  POutMax=[]  IOutMin=[]  IOutMax=[]  DOutMin=[]  DOutMax=[]  NOutMin=[]  NOutMax=[]  SumOutMin=[]  SumOutMax=[]  SaturationOutMin=[]  SaturationOutMax=[]  PParamMin=[]  PParamMax=[]  IParamMin=[]  IParamMax=[]  DParamMin=[]  DParamMax=[]  NParamMin=[]  NParamMax=[]  KbParamMin=[]  KbParamMax=[]  KtParamMin=[]  KtParamMax=[]  KbOutMin=[]  KbOutMax=[]  KtOutMin=[]  KtOutMax=[]  IntegratorOutMin=[]  IntegratorOutMax=[]  FilterOutMin=[]  FilterOutMax=[]  SumI1OutMin=[]  SumI1OutMax=[]  SumI2OutMin=[]  SumI2OutMax=[]  SumI3OutMin=[]  SumI3OutMax=[]  SumI4OutMin=[]  SumI4OutMax=[]  SumDOutMin=[]  SumDOutMax=[]  DifferentiatorOutMin=[]  DifferentiatorOutMax=[]  FilterDiffOutCoefMin=[]  FilterDiffOutCoefMax=[]  ReciprocalOutMin=[]  ReciprocalOutMax=[]  SumDenOutMin=[]  SumDenOutMax=[]  SumNumOutMin=[]  SumNumOutMax=[]  DivideOutMin=[]  DivideOutMax=[]  UdiffTsProdOutMin=[]  UdiffTsProdOutMax=[]  NTsProdOutMin=[]  NTsProdOutMax=[]  UintegralTsProdOutMin=[]  UintegralTsProdOutMax=[]  UngainTsProdOutMin=[]  UngainTsProdOutMax=[]  ClampingZeroOutDataTypeStr=Inherit: Inherit via back propagation  ClampingZeroOutMin=[]  ClampingZeroOutMax=[]  FilterDenConstantOutDataTypeStr=Inherit: Inherit via back propagation  FilterDenConstantOutMin=[]  FilterDenConstantOutMax=[]  PCopyOutDataTypeStr=Inherit: Inherit via back propagation  PCopyOutMin=[]  PCopyOutMax=[]  NCopyOutDataTypeStr=Inherit: Inherit via back propagation  NCopyOutMin=[]  NCopyOutMax=[]  IntegratorContinuousStateAttributes=''  IntegratorStateMustResolveToSignalObject=off  IntegratorRTWStateStorageClass=Auto  FilterContinuousStateAttributes=''  FilterStateMustResolveToSignalObject=off  FilterRTWStateStorageClass=Auto  ParallelPVariant=InternalParameters  IdealPVariant=Disabled  IVariant=InternalParameters  DVariant=Disabled  IntegratorVariant=Continuous  SatVariant=Disabled  AWVariant=Passthrough  PCopyVariant=Disabled  TRVariant=Disabled  FdbkBlocksVariant=Forward  IdealPFdbkVariant=Disabled  SatFdbkVariant=Disabled  DerivativeFilterVariant=Disabled  NVariant=Disabled  NCopyVariant=Disabled_SignalSpec  FilterICVariant=Disabled  IntegratorICVariant=InternalICs  ExternalResetVariant=Disabled  TRSumVariant=Passthrough  SumFdbkVariant=Disabled  SumVariant=Sum_PI  TsampFilterVariant=InternalTs  TsampNgainVariant=Passthrough  TsampIntegralVariant=Disabled_SignalSpec  ExternalSaturationOutDataTypeStr=Inherit: Same as second input  DerivativeSourceVariant=Disabled  PreIntVariant=InternalPreInt
  PID Controller3 : slpidlib/PID Controller  Commented=on  Controller=PI  Form=Parallel  TimeDomain=Continuous-time  UseExternalTs=off  SampleTime=-1  IntegratorMethod=Forward Euler  FilterMethod=Forward Euler  ControllerParametersSource=internal  P=0  I=238.210092745493  UseKiTs=off  D=0  UseExternalDerivativeSource=off  N=100  UseFilter=on  TunerSelectOption=Transfer Function Based (PID Tuner App)  InitialConditionSource=internal  InitialConditionForIntegrator=7000  InitialConditionForFilter=0  DifferentiatorICPrevScaledInput=0  ExternalReset=none  TrackingMode=off  Kt=1  LimitOutput=off  SatLimitsSource=internal  UpperSaturationLimit=inf  LowerSaturationLimit=-inf  LinearizeAsGain=on  AntiWindupMode=none  Kb=1  LimitIntegrator=off  UpperIntegratorSaturationLimit=inf  LowerIntegratorSaturationLimit=-inf  POutMin=[]  POutMax=[]  IOutMin=[]  IOutMax=[]  DOutMin=[]  DOutMax=[]  NOutMin=[]  NOutMax=[]  SumOutMin=[]  SumOutMax=[]  SaturationOutMin=[]  SaturationOutMax=[]  PParamMin=[]  PParamMax=[]  IParamMin=[]  IParamMax=[]  DParamMin=[]  DParamMax=[]  NParamMin=[]  NParamMax=[]  KbParamMin=[]  KbParamMax=[]  KtParamMin=[]  KtParamMax=[]  KbOutMin=[]  KbOutMax=[]  KtOutMin=[]  KtOutMax=[]  IntegratorOutMin=[]  IntegratorOutMax=[]  FilterOutMin=[]  FilterOutMax=[]  SumI1OutMin=[]  SumI1OutMax=[]  SumI2OutMin=[]  SumI2OutMax=[]  SumI3OutMin=[]  SumI3OutMax=[]  SumI4OutMin=[]  SumI4OutMax=[]  SumDOutMin=[]  SumDOutMax=[]  DifferentiatorOutMin=[]  DifferentiatorOutMax=[]  FilterDiffOutCoefMin=[]  FilterDiffOutCoefMax=[]  ReciprocalOutMin=[]  ReciprocalOutMax=[]  SumDenOutMin=[]  SumDenOutMax=[]  SumNumOutMin=[]  SumNumOutMax=[]  DivideOutMin=[]  DivideOutMax=[]  UdiffTsProdOutMin=[]  UdiffTsProdOutMax=[]  NTsProdOutMin=[]  NTsProdOutMax=[]  UintegralTsProdOutMin=[]  UintegralTsProdOutMax=[]  UngainTsProdOutMin=[]  UngainTsProdOutMax=[]  ClampingZeroOutDataTypeStr=Inherit: Inherit via back propagation  ClampingZeroOutMin=[]  ClampingZeroOutMax=[]  FilterDenConstantOutDataTypeStr=Inherit: Inherit via back propagation  FilterDenConstantOutMin=[]  FilterDenConstantOutMax=[]  PCopyOutDataTypeStr=Inherit: Inherit via back propagation  PCopyOutMin=[]  PCopyOutMax=[]  NCopyOutDataTypeStr=Inherit: Inherit via back propagation  NCopyOutMin=[]  NCopyOutMax=[]  IntegratorContinuousStateAttributes=''  IntegratorStateMustResolveToSignalObject=off  IntegratorRTWStateStorageClass=Auto  FilterContinuousStateAttributes=''  FilterStateMustResolveToSignalObject=off  FilterRTWStateStorageClass=Auto  ParallelPVariant=InternalParameters  IdealPVariant=Disabled  IVariant=InternalParameters  DVariant=Disabled  IntegratorVariant=Continuous  SatVariant=Disabled  AWVariant=Passthrough  PCopyVariant=Disabled  TRVariant=Disabled  FdbkBlocksVariant=Forward  IdealPFdbkVariant=Disabled  SatFdbkVariant=Disabled  DerivativeFilterVariant=Disabled  NVariant=Disabled  NCopyVariant=Disabled_SignalSpec  FilterICVariant=Disabled  IntegratorICVariant=InternalICs  ExternalResetVariant=Disabled  TRSumVariant=Passthrough  SumFdbkVariant=Disabled  SumVariant=Sum_PI  TsampFilterVariant=InternalTs  TsampNgainVariant=Passthrough  TsampIntegralVariant=Disabled_SignalSpec  ExternalSaturationOutDataTypeStr=Inherit: Same as second input  DerivativeSourceVariant=Disabled  PreIntVariant=InternalPreInt
  PID Controller4 : slpidlib/PID Controller  Commented=on  Controller=PI  Form=Parallel  TimeDomain=Continuous-time  UseExternalTs=off  SampleTime=-1  IntegratorMethod=Forward Euler  FilterMethod=Forward Euler  ControllerParametersSource=internal  P=-3.92224386090131  I=-5.88659038556754  UseKiTs=off  D=0  UseExternalDerivativeSource=off  N=100  UseFilter=on  TunerSelectOption=Transfer Function Based (PID Tuner App)  InitialConditionSource=internal  InitialConditionForIntegrator=5.056  InitialConditionForFilter=0  DifferentiatorICPrevScaledInput=0  ExternalReset=none  TrackingMode=off  Kt=1  LimitOutput=off  SatLimitsSource=internal  UpperSaturationLimit=inf  LowerSaturationLimit=-inf  LinearizeAsGain=on  AntiWindupMode=none  Kb=1  LimitIntegrator=off  UpperIntegratorSaturationLimit=inf  LowerIntegratorSaturationLimit=-inf  POutMin=[]  POutMax=[]  IOutMin=[]  IOutMax=[]  DOutMin=[]  DOutMax=[]  NOutMin=[]  NOutMax=[]  SumOutMin=[]  SumOutMax=[]  SaturationOutMin=[]  SaturationOutMax=[]  PParamMin=[]  PParamMax=[]  IParamMin=[]  IParamMax=[]  DParamMin=[]  DParamMax=[]  NParamMin=[]  NParamMax=[]  KbParamMin=[]  KbParamMax=[]  KtParamMin=[]  KtParamMax=[]  KbOutMin=[]  KbOutMax=[]  KtOutMin=[]  KtOutMax=[]  IntegratorOutMin=[]  IntegratorOutMax=[]  FilterOutMin=[]  FilterOutMax=[]  SumI1OutMin=[]  SumI1OutMax=[]  SumI2OutMin=[]  SumI2OutMax=[]  SumI3OutMin=[]  SumI3OutMax=[]  SumI4OutMin=[]  SumI4OutMax=[]  SumDOutMin=[]  SumDOutMax=[]  DifferentiatorOutMin=[]  DifferentiatorOutMax=[]  FilterDiffOutCoefMin=[]  FilterDiffOutCoefMax=[]  ReciprocalOutMin=[]  ReciprocalOutMax=[]  SumDenOutMin=[]  SumDenOutMax=[]  SumNumOutMin=[]  SumNumOutMax=[]  DivideOutMin=[]  DivideOutMax=[]  UdiffTsProdOutMin=[]  UdiffTsProdOutMax=[]  NTsProdOutMin=[]  NTsProdOutMax=[]  UintegralTsProdOutMin=[]  UintegralTsProdOutMax=[]  UngainTsProdOutMin=[]  UngainTsProdOutMax=[]  ClampingZeroOutDataTypeStr=Inherit: Inherit via back propagation  ClampingZeroOutMin=[]  ClampingZeroOutMax=[]  FilterDenConstantOutDataTypeStr=Inherit: Inherit via back propagation  FilterDenConstantOutMin=[]  FilterDenConstantOutMax=[]  PCopyOutDataTypeStr=Inherit: Inherit via back propagation  PCopyOutMin=[]  PCopyOutMax=[]  NCopyOutDataTypeStr=Inherit: Inherit via back propagation  NCopyOutMin=[]  NCopyOutMax=[]  IntegratorContinuousStateAttributes=''  IntegratorStateMustResolveToSignalObject=off  IntegratorRTWStateStorageClass=Auto  FilterContinuousStateAttributes=''  FilterStateMustResolveToSignalObject=off  FilterRTWStateStorageClass=Auto  ParallelPVariant=InternalParameters  IdealPVariant=Disabled  IVariant=InternalParameters  DVariant=Disabled  IntegratorVariant=Continuous  SatVariant=Disabled  AWVariant=Passthrough  PCopyVariant=Disabled  TRVariant=Disabled  FdbkBlocksVariant=Forward  IdealPFdbkVariant=Disabled  SatFdbkVariant=Disabled  DerivativeFilterVariant=Disabled  NVariant=Disabled  NCopyVariant=Disabled_SignalSpec  FilterICVariant=Disabled  IntegratorICVariant=InternalICs  ExternalResetVariant=Disabled  TRSumVariant=Passthrough  SumFdbkVariant=Disabled  SumVariant=Sum_PI  TsampFilterVariant=InternalTs  TsampNgainVariant=Passthrough  TsampIntegralVariant=Disabled_SignalSpec  ExternalSaturationOutDataTypeStr=Inherit: Same as second input  DerivativeSourceVariant=Disabled  PreIntVariant=InternalPreInt
  PID Controller5 : slpidlib/PID Controller  Commented=on  Controller=PI  Form=Parallel  TimeDomain=Continuous-time  UseExternalTs=off  SampleTime=-1  IntegratorMethod=Forward Euler  FilterMethod=Forward Euler  ControllerParametersSource=internal  P=4.61666206251897  I=6.04498234609336  UseKiTs=off  D=0  UseExternalDerivativeSource=off  N=100  UseFilter=on  TunerSelectOption=Transfer Function Based (PID Tuner App)  InitialConditionSource=internal  InitialConditionForIntegrator=5.057  InitialConditionForFilter=0  DifferentiatorICPrevScaledInput=0  ExternalReset=none  TrackingMode=off  Kt=1  LimitOutput=off  SatLimitsSource=internal  UpperSaturationLimit=inf  LowerSaturationLimit=-inf  LinearizeAsGain=on  AntiWindupMode=none  Kb=1  LimitIntegrator=off  UpperIntegratorSaturationLimit=inf  LowerIntegratorSaturationLimit=-inf  POutMin=[]  POutMax=[]  IOutMin=[]  IOutMax=[]  DOutMin=[]  DOutMax=[]  NOutMin=[]  NOutMax=[]  SumOutMin=[]  SumOutMax=[]  SaturationOutMin=[]  SaturationOutMax=[]  PParamMin=[]  PParamMax=[]  IParamMin=[]  IParamMax=[]  DParamMin=[]  DParamMax=[]  NParamMin=[]  NParamMax=[]  KbParamMin=[]  KbParamMax=[]  KtParamMin=[]  KtParamMax=[]  KbOutMin=[]  KbOutMax=[]  KtOutMin=[]  KtOutMax=[]  IntegratorOutMin=[]  IntegratorOutMax=[]  FilterOutMin=[]  FilterOutMax=[]  SumI1OutMin=[]  SumI1OutMax=[]  SumI2OutMin=[]  SumI2OutMax=[]  SumI3OutMin=[]  SumI3OutMax=[]  SumI4OutMin=[]  SumI4OutMax=[]  SumDOutMin=[]  SumDOutMax=[]  DifferentiatorOutMin=[]  DifferentiatorOutMax=[]  FilterDiffOutCoefMin=[]  FilterDiffOutCoefMax=[]  ReciprocalOutMin=[]  ReciprocalOutMax=[]  SumDenOutMin=[]  SumDenOutMax=[]  SumNumOutMin=[]  SumNumOutMax=[]  DivideOutMin=[]  DivideOutMax=[]  UdiffTsProdOutMin=[]  UdiffTsProdOutMax=[]  NTsProdOutMin=[]  NTsProdOutMax=[]  UintegralTsProdOutMin=[]  UintegralTsProdOutMax=[]  UngainTsProdOutMin=[]  UngainTsProdOutMax=[]  ClampingZeroOutDataTypeStr=Inherit: Inherit via back propagation  ClampingZeroOutMin=[]  ClampingZeroOutMax=[]  FilterDenConstantOutDataTypeStr=Inherit: Inherit via back propagation  FilterDenConstantOutMin=[]  FilterDenConstantOutMax=[]  PCopyOutDataTypeStr=Inherit: Inherit via back propagation  PCopyOutMin=[]  PCopyOutMax=[]  NCopyOutDataTypeStr=Inherit: Inherit via back propagation  NCopyOutMin=[]  NCopyOutMax=[]  IntegratorContinuousStateAttributes=''  IntegratorStateMustResolveToSignalObject=off  IntegratorRTWStateStorageClass=Auto  FilterContinuousStateAttributes=''  FilterStateMustResolveToSignalObject=off  FilterRTWStateStorageClass=Auto  ParallelPVariant=InternalParameters  IdealPVariant=Disabled  IVariant=InternalParameters  DVariant=Disabled  IntegratorVariant=Continuous  SatVariant=Disabled  AWVariant=Passthrough  PCopyVariant=Disabled  TRVariant=Disabled  FdbkBlocksVariant=Forward  IdealPFdbkVariant=Disabled  SatFdbkVariant=Disabled  DerivativeFilterVariant=Disabled  NVariant=Disabled  NCopyVariant=Disabled_SignalSpec  FilterICVariant=Disabled  IntegratorICVariant=InternalICs  ExternalResetVariant=Disabled  TRSumVariant=Passthrough  SumFdbkVariant=Disabled  SumVariant=Sum_PI  TsampFilterVariant=InternalTs  TsampNgainVariant=Passthrough  TsampIntegralVariant=Disabled_SignalSpec  ExternalSaturationOutDataTypeStr=Inherit: Same as second input  DerivativeSourceVariant=Disabled  PreIntVariant=InternalPreInt
  PID Controller6 : slpidlib/PID Controller  Commented=on  Controller=PI  Form=Parallel  TimeDomain=Continuous-time  UseExternalTs=off  SampleTime=-1  IntegratorMethod=Forward Euler  FilterMethod=Forward Euler  ControllerParametersSource=internal  P=0  I=1436.64485863515  UseKiTs=off  D=0  UseExternalDerivativeSource=off  N=100  UseFilter=on  TunerSelectOption=Transfer Function Based (PID Tuner App)  InitialConditionSource=internal  InitialConditionForIntegrator=1170  InitialConditionForFilter=0  DifferentiatorICPrevScaledInput=0  ExternalReset=none  TrackingMode=off  Kt=1  LimitOutput=off  SatLimitsSource=internal  UpperSaturationLimit=inf  LowerSaturationLimit=-inf  LinearizeAsGain=on  AntiWindupMode=none  Kb=1  LimitIntegrator=off  UpperIntegratorSaturationLimit=inf  LowerIntegratorSaturationLimit=-inf  POutMin=[]  POutMax=[]  IOutMin=[]  IOutMax=[]  DOutMin=[]  DOutMax=[]  NOutMin=[]  NOutMax=[]  SumOutMin=[]  SumOutMax=[]  SaturationOutMin=[]  SaturationOutMax=[]  PParamMin=[]  PParamMax=[]  IParamMin=[]  IParamMax=[]  DParamMin=[]  DParamMax=[]  NParamMin=[]  NParamMax=[]  KbParamMin=[]  KbParamMax=[]  KtParamMin=[]  KtParamMax=[]  KbOutMin=[]  KbOutMax=[]  KtOutMin=[]  KtOutMax=[]  IntegratorOutMin=[]  IntegratorOutMax=[]  FilterOutMin=[]  FilterOutMax=[]  SumI1OutMin=[]  SumI1OutMax=[]  SumI2OutMin=[]  SumI2OutMax=[]  SumI3OutMin=[]  SumI3OutMax=[]  SumI4OutMin=[]  SumI4OutMax=[]  SumDOutMin=[]  SumDOutMax=[]  DifferentiatorOutMin=[]  DifferentiatorOutMax=[]  FilterDiffOutCoefMin=[]  FilterDiffOutCoefMax=[]  ReciprocalOutMin=[]  ReciprocalOutMax=[]  SumDenOutMin=[]  SumDenOutMax=[]  SumNumOutMin=[]  SumNumOutMax=[]  DivideOutMin=[]  DivideOutMax=[]  UdiffTsProdOutMin=[]  UdiffTsProdOutMax=[]  NTsProdOutMin=[]  NTsProdOutMax=[]  UintegralTsProdOutMin=[]  UintegralTsProdOutMax=[]  UngainTsProdOutMin=[]  UngainTsProdOutMax=[]  ClampingZeroOutDataTypeStr=Inherit: Inherit via back propagation  ClampingZeroOutMin=[]  ClampingZeroOutMax=[]  FilterDenConstantOutDataTypeStr=Inherit: Inherit via back propagation  FilterDenConstantOutMin=[]  FilterDenConstantOutMax=[]  PCopyOutDataTypeStr=Inherit: Inherit via back propagation  PCopyOutMin=[]  PCopyOutMax=[]  NCopyOutDataTypeStr=Inherit: Inherit via back propagation  NCopyOutMin=[]  NCopyOutMax=[]  IntegratorContinuousStateAttributes=''  IntegratorStateMustResolveToSignalObject=off  IntegratorRTWStateStorageClass=Auto  FilterContinuousStateAttributes=''  FilterStateMustResolveToSignalObject=off  FilterRTWStateStorageClass=Auto  ParallelPVariant=InternalParameters  IdealPVariant=Disabled  IVariant=InternalParameters  DVariant=Disabled  IntegratorVariant=Continuous  SatVariant=Disabled  AWVariant=Passthrough  PCopyVariant=Disabled  TRVariant=Disabled  FdbkBlocksVariant=Forward  IdealPFdbkVariant=Disabled  SatFdbkVariant=Disabled  DerivativeFilterVariant=Disabled  NVariant=Disabled  NCopyVariant=Disabled_SignalSpec  FilterICVariant=Disabled  IntegratorICVariant=InternalICs  ExternalResetVariant=Disabled  TRSumVariant=Passthrough  SumFdbkVariant=Disabled  SumVariant=Sum_PI  TsampFilterVariant=InternalTs  TsampNgainVariant=Passthrough  TsampIntegralVariant=Disabled_SignalSpec  ExternalSaturationOutDataTypeStr=Inherit: Same as second input  DerivativeSourceVariant=Disabled  PreIntVariant=InternalPreInt
  PID Controller7 : slpidlib/PID Controller  Commented=on  Controller=PI  Form=Parallel  TimeDomain=Continuous-time  UseExternalTs=off  SampleTime=-1  IntegratorMethod=Forward Euler  FilterMethod=Forward Euler  ControllerParametersSource=internal  P=-6.25982057355693  I=-4.98960589901713  UseKiTs=off  D=0  UseExternalDerivativeSource=off  N=100  UseFilter=on  TunerSelectOption=Transfer Function Based (PID Tuner App)  InitialConditionSource=internal  InitialConditionForIntegrator=2.253  InitialConditionForFilter=0  DifferentiatorICPrevScaledInput=0  ExternalReset=none  TrackingMode=off  Kt=1  LimitOutput=off  SatLimitsSource=internal  UpperSaturationLimit=inf  LowerSaturationLimit=-inf  LinearizeAsGain=on  AntiWindupMode=none  Kb=1  LimitIntegrator=off  UpperIntegratorSaturationLimit=inf  LowerIntegratorSaturationLimit=-inf  POutMin=[]  POutMax=[]  IOutMin=[]  IOutMax=[]  DOutMin=[]  DOutMax=[]  NOutMin=[]  NOutMax=[]  SumOutMin=[]  SumOutMax=[]  SaturationOutMin=[]  SaturationOutMax=[]  PParamMin=[]  PParamMax=[]  IParamMin=[]  IParamMax=[]  DParamMin=[]  DParamMax=[]  NParamMin=[]  NParamMax=[]  KbParamMin=[]  KbParamMax=[]  KtParamMin=[]  KtParamMax=[]  KbOutMin=[]  KbOutMax=[]  KtOutMin=[]  KtOutMax=[]  IntegratorOutMin=[]  IntegratorOutMax=[]  FilterOutMin=[]  FilterOutMax=[]  SumI1OutMin=[]  SumI1OutMax=[]  SumI2OutMin=[]  SumI2OutMax=[]  SumI3OutMin=[]  SumI3OutMax=[]  SumI4OutMin=[]  SumI4OutMax=[]  SumDOutMin=[]  SumDOutMax=[]  DifferentiatorOutMin=[]  DifferentiatorOutMax=[]  FilterDiffOutCoefMin=[]  FilterDiffOutCoefMax=[]  ReciprocalOutMin=[]  ReciprocalOutMax=[]  SumDenOutMin=[]  SumDenOutMax=[]  SumNumOutMin=[]  SumNumOutMax=[]  DivideOutMin=[]  DivideOutMax=[]  UdiffTsProdOutMin=[]  UdiffTsProdOutMax=[]  NTsProdOutMin=[]  NTsProdOutMax=[]  UintegralTsProdOutMin=[]  UintegralTsProdOutMax=[]  UngainTsProdOutMin=[]  UngainTsProdOutMax=[]  ClampingZeroOutDataTypeStr=Inherit: Inherit via back propagation  ClampingZeroOutMin=[]  ClampingZeroOutMax=[]  FilterDenConstantOutDataTypeStr=Inherit: Inherit via back propagation  FilterDenConstantOutMin=[]  FilterDenConstantOutMax=[]  PCopyOutDataTypeStr=Inherit: Inherit via back propagation  PCopyOutMin=[]  PCopyOutMax=[]  NCopyOutDataTypeStr=Inherit: Inherit via back propagation  NCopyOutMin=[]  NCopyOutMax=[]  IntegratorContinuousStateAttributes=''  IntegratorStateMustResolveToSignalObject=off  IntegratorRTWStateStorageClass=Auto  FilterContinuousStateAttributes=''  FilterStateMustResolveToSignalObject=off  FilterRTWStateStorageClass=Auto  ParallelPVariant=InternalParameters  IdealPVariant=Disabled  IVariant=InternalParameters  DVariant=Disabled  IntegratorVariant=Continuous  SatVariant=Disabled  AWVariant=Passthrough  PCopyVariant=Disabled  TRVariant=Disabled  FdbkBlocksVariant=Forward  IdealPFdbkVariant=Disabled  SatFdbkVariant=Disabled  DerivativeFilterVariant=Disabled  NVariant=Disabled  NCopyVariant=Disabled_SignalSpec  FilterICVariant=Disabled  IntegratorICVariant=InternalICs  ExternalResetVariant=Disabled  TRSumVariant=Passthrough  SumFdbkVariant=Disabled  SumVariant=Sum_PI  TsampFilterVariant=InternalTs  TsampNgainVariant=Passthrough  TsampIntegralVariant=Disabled_SignalSpec  ExternalSaturationOutDataTypeStr=Inherit: Same as second input  DerivativeSourceVariant=Disabled  PreIntVariant=InternalPreInt
  PID Controller8 : slpidlib/PID Controller  Commented=on  Controller=PI  Form=Parallel  TimeDomain=Continuous-time  UseExternalTs=off  SampleTime=-1  IntegratorMethod=Forward Euler  FilterMethod=Forward Euler  ControllerParametersSource=internal  P=-7.51009745497026  I=-8.10801960774173  UseKiTs=off  D=0  UseExternalDerivativeSource=off  N=100  UseFilter=on  TunerSelectOption=Transfer Function Based (PID Tuner App)  InitialConditionSource=internal  InitialConditionForIntegrator=2.253  InitialConditionForFilter=0  DifferentiatorICPrevScaledInput=0  ExternalReset=none  TrackingMode=off  Kt=1  LimitOutput=off  SatLimitsSource=internal  UpperSaturationLimit=inf  LowerSaturationLimit=-inf  LinearizeAsGain=on  AntiWindupMode=none  Kb=1  LimitIntegrator=off  UpperIntegratorSaturationLimit=inf  LowerIntegratorSaturationLimit=-inf  POutMin=[]  POutMax=[]  IOutMin=[]  IOutMax=[]  DOutMin=[]  DOutMax=[]  NOutMin=[]  NOutMax=[]  SumOutMin=[]  SumOutMax=[]  SaturationOutMin=[]  SaturationOutMax=[]  PParamMin=[]  PParamMax=[]  IParamMin=[]  IParamMax=[]  DParamMin=[]  DParamMax=[]  NParamMin=[]  NParamMax=[]  KbParamMin=[]  KbParamMax=[]  KtParamMin=[]  KtParamMax=[]  KbOutMin=[]  KbOutMax=[]  KtOutMin=[]  KtOutMax=[]  IntegratorOutMin=[]  IntegratorOutMax=[]  FilterOutMin=[]  FilterOutMax=[]  SumI1OutMin=[]  SumI1OutMax=[]  SumI2OutMin=[]  SumI2OutMax=[]  SumI3OutMin=[]  SumI3OutMax=[]  SumI4OutMin=[]  SumI4OutMax=[]  SumDOutMin=[]  SumDOutMax=[]  DifferentiatorOutMin=[]  DifferentiatorOutMax=[]  FilterDiffOutCoefMin=[]  FilterDiffOutCoefMax=[]  ReciprocalOutMin=[]  ReciprocalOutMax=[]  SumDenOutMin=[]  SumDenOutMax=[]  SumNumOutMin=[]  SumNumOutMax=[]  DivideOutMin=[]  DivideOutMax=[]  UdiffTsProdOutMin=[]  UdiffTsProdOutMax=[]  NTsProdOutMin=[]  NTsProdOutMax=[]  UintegralTsProdOutMin=[]  UintegralTsProdOutMax=[]  UngainTsProdOutMin=[]  UngainTsProdOutMax=[]  ClampingZeroOutDataTypeStr=Inherit: Inherit via back propagation  ClampingZeroOutMin=[]  ClampingZeroOutMax=[]  FilterDenConstantOutDataTypeStr=Inherit: Inherit via back propagation  FilterDenConstantOutMin=[]  FilterDenConstantOutMax=[]  PCopyOutDataTypeStr=Inherit: Inherit via back propagation  PCopyOutMin=[]  PCopyOutMax=[]  NCopyOutDataTypeStr=Inherit: Inherit via back propagation  NCopyOutMin=[]  NCopyOutMax=[]  IntegratorContinuousStateAttributes=''  IntegratorStateMustResolveToSignalObject=off  IntegratorRTWStateStorageClass=Auto  FilterContinuousStateAttributes=''  FilterStateMustResolveToSignalObject=off  FilterRTWStateStorageClass=Auto  ParallelPVariant=InternalParameters  IdealPVariant=Disabled  IVariant=InternalParameters  DVariant=Disabled  IntegratorVariant=Continuous  SatVariant=Disabled  AWVariant=Passthrough  PCopyVariant=Disabled  TRVariant=Disabled  FdbkBlocksVariant=Forward  IdealPFdbkVariant=Disabled  SatFdbkVariant=Disabled  DerivativeFilterVariant=Disabled  NVariant=Disabled  NCopyVariant=Disabled_SignalSpec  FilterICVariant=Disabled  IntegratorICVariant=InternalICs  ExternalResetVariant=Disabled  TRSumVariant=Passthrough  SumFdbkVariant=Disabled  SumVariant=Sum_PI  TsampFilterVariant=InternalTs  TsampNgainVariant=Passthrough  TsampIntegralVariant=Disabled_SignalSpec  ExternalSaturationOutDataTypeStr=Inherit: Same as second input  DerivativeSourceVariant=Disabled  PreIntVariant=InternalPreInt
  PID Controller9 : slpidlib/PID Controller  Commented=on  Controller=PI  Form=Parallel  TimeDomain=Continuous-time  UseExternalTs=off  SampleTime=-1  IntegratorMethod=Forward Euler  FilterMethod=Forward Euler  ControllerParametersSource=internal  P=-6.30860731604003  I=-0.696651988921177  UseKiTs=off  D=0  UseExternalDerivativeSource=off  N=100  UseFilter=on  TunerSelectOption=Transfer Function Based (PID Tuner App)  InitialConditionSource=internal  InitialConditionForIntegrator=2.253  InitialConditionForFilter=0  DifferentiatorICPrevScaledInput=0  ExternalReset=none  TrackingMode=off  Kt=1  LimitOutput=off  SatLimitsSource=internal  UpperSaturationLimit=inf  LowerSaturationLimit=-inf  LinearizeAsGain=on  AntiWindupMode=none  Kb=1  LimitIntegrator=off  UpperIntegratorSaturationLimit=inf  LowerIntegratorSaturationLimit=-inf  POutMin=[]  POutMax=[]  IOutMin=[]  IOutMax=[]  DOutMin=[]  DOutMax=[]  NOutMin=[]  NOutMax=[]  SumOutMin=[]  SumOutMax=[]  SaturationOutMin=[]  SaturationOutMax=[]  PParamMin=[]  PParamMax=[]  IParamMin=[]  IParamMax=[]  DParamMin=[]  DParamMax=[]  NParamMin=[]  NParamMax=[]  KbParamMin=[]  KbParamMax=[]  KtParamMin=[]  KtParamMax=[]  KbOutMin=[]  KbOutMax=[]  KtOutMin=[]  KtOutMax=[]  IntegratorOutMin=[]  IntegratorOutMax=[]  FilterOutMin=[]  FilterOutMax=[]  SumI1OutMin=[]  SumI1OutMax=[]  SumI2OutMin=[]  SumI2OutMax=[]  SumI3OutMin=[]  SumI3OutMax=[]  SumI4OutMin=[]  SumI4OutMax=[]  SumDOutMin=[]  SumDOutMax=[]  DifferentiatorOutMin=[]  DifferentiatorOutMax=[]  FilterDiffOutCoefMin=[]  FilterDiffOutCoefMax=[]  ReciprocalOutMin=[]  ReciprocalOutMax=[]  SumDenOutMin=[]  SumDenOutMax=[]  SumNumOutMin=[]  SumNumOutMax=[]  DivideOutMin=[]  DivideOutMax=[]  UdiffTsProdOutMin=[]  UdiffTsProdOutMax=[]  NTsProdOutMin=[]  NTsProdOutMax=[]  UintegralTsProdOutMin=[]  UintegralTsProdOutMax=[]  UngainTsProdOutMin=[]  UngainTsProdOutMax=[]  ClampingZeroOutDataTypeStr=Inherit: Inherit via back propagation  ClampingZeroOutMin=[]  ClampingZeroOutMax=[]  FilterDenConstantOutDataTypeStr=Inherit: Inherit via back propagation  FilterDenConstantOutMin=[]  FilterDenConstantOutMax=[]  PCopyOutDataTypeStr=Inherit: Inherit via back propagation  PCopyOutMin=[]  PCopyOutMax=[]  NCopyOutDataTypeStr=Inherit: Inherit via back propagation  NCopyOutMin=[]  NCopyOutMax=[]  IntegratorContinuousStateAttributes=''  IntegratorStateMustResolveToSignalObject=off  IntegratorRTWStateStorageClass=Auto  FilterContinuousStateAttributes=''  FilterStateMustResolveToSignalObject=off  FilterRTWStateStorageClass=Auto  ParallelPVariant=InternalParameters  IdealPVariant=Disabled  IVariant=InternalParameters  DVariant=Disabled  IntegratorVariant=Continuous  SatVariant=Disabled  AWVariant=Passthrough  PCopyVariant=Disabled  TRVariant=Disabled  FdbkBlocksVariant=Forward  IdealPFdbkVariant=Disabled  SatFdbkVariant=Disabled  DerivativeFilterVariant=Disabled  NVariant=Disabled  NCopyVariant=Disabled_SignalSpec  FilterICVariant=Disabled  IntegratorICVariant=InternalICs  ExternalResetVariant=Disabled  TRSumVariant=Passthrough  SumFdbkVariant=Disabled  SumVariant=Sum_PI  TsampFilterVariant=InternalTs  TsampNgainVariant=Passthrough  TsampIntegralVariant=Disabled_SignalSpec  ExternalSaturationOutDataTypeStr=Inherit: Same as second input  DerivativeSourceVariant=Disabled  PreIntVariant=InternalPreInt
  "Pressure, P" : Scope
  "Q, PE" : Scope
  "Q, PE, 14" : Scope  Commented=on
  "Q, Pe-1" : Scope
  "Q, RE, 4" : Scope
  "Q, RE-1" : Scope  Commented=on
  R-101 : S-Function  FunctionName=CSTR  SFunctionDeploymentMode=off  EnableBusSupport=off
  "R-101, C out" : Scope
  "R-101, C:IN,OUT" : Scope  NumInputPorts=2
  "R-101, Level" : Scope
  "R-101, Volume" : Scope
  "R-101, Volume+height" : Scope  NumInputPorts=2
  R-201 : S-Function  Commented=on  FunctionName=Alkalinelysis  SFunctionDeploymentMode=off  EnableBusSupport=off
  "R-201, C,byproduct" : Scope  Commented=on  NumInputPorts=2
  "R-201, C,x" : Scope  Commented=on  NumInputPorts=2
  "R-201, Length " : Scope  Commented=on
  "R-201, Volume" : Scope  Commented=on
  "R-201, Volume+length" : Scope  Commented=on  NumInputPorts=2
  R-301 : S-Function  Commented=on  FunctionName=Linearization  SFunctionDeploymentMode=off  EnableBusSupport=off
  "R-301, C IN/OUT2" : Scope  Commented=on  NumInputPorts=2
  R-401 : S-Function  Commented=on  FunctionName=IVT  SFunctionDeploymentMode=off  EnableBusSupport=off
  "R-401, C IN/OUT1" : Scope  Commented=on  NumInputPorts=2
  R-402 : S-Function  Commented=on  FunctionName=Degradation_reactor  SFunctionDeploymentMode=off  EnableBusSupport=off
  "R-402, C IN/OUT2" : Scope  Commented=on  NumInputPorts=2
  "Resuspension, IN/OUT1" : Scope  Commented=on  NumInputPorts=2
  Scope{,1..101,103,106..125,127} (124 alike) : Scope  Commented=on
  Scope{102,104..105,128} (4 alike) : Scope
  Subtract : Sum  Inputs=+-
  Subtract1 : Sum  Inputs=+-
  Subtract{3..15} (13 alike) : Sum  Commented=on  Inputs=+-
  Subtract2 : Sum  Inputs=+-
  T-101 : S-Function  FunctionName=T_101  SFunctionDeploymentMode=off  EnableBusSupport=off
  T-101 volume : Scope
  "T-101, out" : Scope
  T-205 : S-Function  Commented=on  FunctionName=T_205  SFunctionDeploymentMode=off  EnableBusSupport=off
  T-302 : S-Function  Commented=on  FunctionName=T_302  SFunctionDeploymentMode=off  EnableBusSupport=off
  T-402 : S-Function  Commented=on  FunctionName=T_402  SFunctionDeploymentMode=off  EnableBusSupport=off
  T-501 : S-Function  Commented=on  FunctionName=T_501  SFunctionDeploymentMode=off  EnableBusSupport=off
  "Tank-101, IN/OUT" : Scope  NumInputPorts=2
  "Tank-205, IN/OUT1" : Scope  Commented=on  NumInputPorts=2
  "Total flow, out" : Scope  Commented=on
  UF-101 : MATLAB Function  TreatAsAtomicUnit=on
  "UF-101, C, R/P" : Scope  NumInputPorts=2
  "UF-101, C, R/P1" : Scope  Commented=on  NumInputPorts=2
  "UF-101, Q, R/P" : Scope  NumInputPorts=2
  "UF-101, Q, R/P1" : Scope  Commented=on  NumInputPorts=2
  UF-201 : MATLAB Function  Commented=on  TreatAsAtomicUnit=on
  "UF-201, C, R/P2" : Scope  Commented=on  NumInputPorts=2
  "UF-201, Q, R/P2" : Scope  Commented=on  NumInputPorts=2
  UF-301 : MATLAB Function  Commented=on  TreatAsAtomicUnit=on
  UF-401 : MATLAB Function  Commented=on  TreatAsAtomicUnit=on
  VSP-101 : MATLAB Function  TreatAsAtomicUnit=on
  VSP-204 : MATLAB Function  Commented=on  TreatAsAtomicUnit=on
  VSP-301 : MATLAB Function  Commented=on  TreatAsAtomicUnit=on
  VSP-401 : MATLAB Function  Commented=on  TreatAsAtomicUnit=on
  VSP-503 : MATLAB Function  Commented=on  TreatAsAtomicUnit=on
  VSP-504 : MATLAB Function  Commented=on  TreatAsAtomicUnit=on
  wires:
  M-101/1(y) -> Demux2/1
  Mux/1 -> M-101/1(u)
  Demux2/2 -> Mux2/2, Mux71/2  "C, Glu"
  Demux2/1 -> Mux71/1, Mux2/1  "C, X"
  R-101/1 -> Demux/1
  Mux2/1 -> R-101/1
  Demux2/3 -> Mux71/3, Mux2/3  "C, N"
  Demux2/4 -> Mux2/4  "Q, in"
  Demux/5 -> "R-101, Volume+height"/2, "R-101, Level"/1  "Level"
  Mux5/1 -> P/1(u)
  UF-101/1(y) -> Demux1/1
  Mux11/1 -> UF-101/1(u)
  Mux4/1 -> VSP-101/1(u)
  Mux1/1 -> "R-101, C out"/1, Mux11/1  "C, out"
  VSP-101/1(y) -> Demux3/1
  Demux3/1 -> Mux6/1  "Q"
  Mux6/1 -> Mux11/2
  Demux1/1 -> Mux5/1, "Q, PE"/1, "UF-101, Q, R/P"/2, "Q, Pe-1"/1  "Q,PE-1"
  Demux1/2 -> "UF-101, Q, R/P"/1, "Q, RE, 4"/1, Mux79/1, Mux9/1  "Q, RE. 4"
  Demux1/3 -> Mux13/1, Mux79/2, Mux9/2  "C, X, RE"
  Demux1/4 -> Mux13/2  "C, Glu, RE"
  Demux1/5 -> Mux13/3  "C, N, RE"
  Demux1/6 -> Mux10/1  "C, X, PE-1"
  Demux1/7 -> Mux10/2  "C, Glu, PE-1"
  Demux1/8 -> Mux10/3  "C, N, PE-1"
  % Purge/1 -> Mux5/2
  Mux9/1 -> T-101/1
  T-101/1 -> "Tank-101, IN/OUT"/2, Demux4/1
  Delay time/1 -> Delay block/2
  P/1(y) -> Delay block/1, " Q, Recycle"/1  "Q, Recycle [L/h]"
  Delay block/1 -> Mux/1  "Q, Recycle [L/h]"
  R-201/1 -> Demux5/1
  Demux5/5 -> Mux18/4, Mux23/5, Mux82/2  "C, Denaturated plasmid"
  Demux5/3 -> Mux83/2, Mux18/2, Mux23/3  "C, Cell_disrupted"
  Demux5/1 -> "R-201, Volume+length"/1, "R-201, Volume"/1  "V"
  Demux5/6 -> Mux18/5, Mux23/6, Mux82/3  "C, Endotoxin"
  Demux5/4 -> Mux82/1, Mux18/3, Mux23/4  "C, pDNA"
  Demux5/2 -> Mux83/1, Mux18/1, Mux23/2  "C, Cell"
  Mux7/1 -> R-201/1
  Mux18/1 -> "Neutralization, IN/OUT2"/1, "C, alkaline lysis, out"/1
  Demux5/7 -> Mux82/4, Mux18/6, Mux23/7  "C, NaOH"
  Demux5/8 -> "R-201, Volume+length"/2, "R-201, Length "/1  "Length"
  Demux4/1 -> Subtract2/2, Mux21/1, T-101 volume/1  "Q"
  MATLAB Function4/1(y) -> "Resuspension, IN/OUT1"/2, Demux8/1
  Demux4/2 -> Mux21/2  "C"
  Mux22/1 -> "Resuspension, IN/OUT1"/1, MATLAB Function4/1(u)
  Mux21/1 -> "T-101, out"/1, Mux22/1
  NaOH [M]/1 -> Mux22/2
  Demux8/1 -> C,X/1, Mux81/1, "R-201, C,x"/1, Mux7/1  "C, X"
  Demux8/3 -> Scope99/1, Mux81/2, Mux7/4  "C, NaOH"
  Demux8/2 -> Scope97/1, Neutralization,flow IN/OUT1/1, Mux23/1, Mux7/2, Mux7/3  "Q"
  Mux23/1 -> MATLAB Function5/1(u)
  MATLAB Function5/1(y) -> Demux9/1
  Demux9/2 -> Mux24/1  "C, Cell"
  Demux9/3 -> Mux24/2  "C, Cell_disrupted"
  Demux9/4 -> Mux24/3  "C, pDNA"
  Demux9/5 -> Mux24/4  "C, Denaturated plasmid"
  Demux9/6 -> Mux24/5  "C, Endotoxin"
  Demux9/7 -> Mux24/6  "C, NaOH"
  Demux6/8 -> Mux16/6  "C, NaOH, RE-1"
  Mux16/1 -> "UF-201, C, R/P2"/1, "C, RE-1"/1
  Demux6/4 -> Mux16/2  "C, Cell_disrupted, RE-1"
  UF-201/1(y) -> Demux6/1
  Demux6/3 -> Mux16/1  "C, Cell, RE-1"
  Mux15/1 -> Mux19/2
  Demux6/7 -> Mux16/5  "C, Endotoxin, RE-1"
  Demux6/6 -> Mux16/4  "C, Denaturated plasmid, RE-1"
  Mux19/1 -> UF-201/1(u)
  VSP-204/1(y) -> Demux7/1
  Mux12/1 -> VSP-204/1(u)
  Demux6/5 -> Mux16/3  "C, pDNA, RE-1"
  Mux24/1 -> "C, neutralization out"/1, "Neutralization, IN/OUT2"/2, Mux19/1  "C, out"
  Mux17/1 -> "UF-201, C, R/P2"/2, "C, PE, 14"/1
  R-301/1 -> Demux12/1
  Demux12/2 -> Mux88/1, Mux34/1  "C, pDNA"
  CH3CO2K [M]/1 -> Mux23/8
  Demux9/8 -> Mux24/7  "C, CH3CO2K"
  Demux6/9 -> Mux16/7  "C, CH3CO2K, RE-1"
  Demux6/10 -> Mux17/1  "C, Cell, PE"
  Demux6/11 -> Mux17/2  "C, Cell_disrupted, PE"
  Demux6/12 -> Mux20/1, Mux17/3, Mux85/1, Mux27/4  "C, pDNA, PE"
  Demux6/13 -> Mux85/3, Mux27/3, Mux17/4  "C, Denaturated plasmid, PE"
  Demux6/14 -> Mux27/2, Mux85/2, Mux17/5  "C, Endotoxin, PE"
  Demux6/15 -> Mux17/6  "C, NaOH, PE"
  Demux6/16 -> Mux17/7  "C, CH3CO2K, PE"
  Demux10/14 -> Scope19/1
  Demux10/16 -> Scope8/1
  Demux10/2 -> Scope29/1
  Demux10/3 -> Scope30/1
  AEX-201:204/1 -> "Output, AEX-201:204"/1, Demux10/1
  Demux10/10 -> Scope23/1
  Demux10/7 -> Scope26/1
  Demux10/1 -> Scope28/1
  Demux10/11 -> Scope22/1
  Demux10/6 -> Scope5/1
  Demux10/15 -> Scope18/1
  Demux10/12 -> Scope21/1
  Demux10/4 -> Mux84/3, Scope2/1  "C, Denaturated plasmid"
  Demux10/13 -> Scope20/1
  Demux10/8 -> Mux84/2, Scope25/1  "C, Endotoxins"
  Demux10/9 -> Scope24/1
  Demux10/5 -> Scope13/1
  Demux10/17 -> Scope7/1
  Mux27/1 -> "Input, AEX-201:204"/1, AEX-201:204/1
  Mux30/1 -> T-205/1
  Demux11/1 -> Subtract4/2, Mux26/3, Mux29/1  "Q"
  Demux12/3 -> Mux88/2, Mux34/2  "C, linpDNA"
  Demux12/4 -> Mux88/3, Mux34/3  "C, Impurities"
  Demux11/2 -> Mux29/2, "R-301, C IN/OUT2"/1, Mux26/1  "C, pDNA"
  UF-301/1(y) -> Demux13/1
  Demux14/1 -> Mux67/1, Scope44/1, Mux32/1  "Q"
  Mux35/1 -> UF-301/1(u)
  Mux32/1 -> Mux35/2
  Demux14/2 -> Scope110/1, Subtract6/2, Mux32/2, Mux67/2  "P"
  Demux13/2 -> "UF-101, Q, R/P1"/1, Scope34/1  "Q, RE-2"
  Mux31/1 -> VSP-301/1(u)
  Mux33/1 -> "UF-101, C, R/P1"/1, "C, RE-2"/1
  VSP-301/1(y) -> Demux14/1
  Demux12/5 -> Mux88/4, Mux34/4  "C, EcoRI enzyme"
  Demux13/3 -> Mux33/1  "C, pDNA, RE-2"
  Demux13/4 -> Mux33/2  "C, linpDNA, RE-2"
  Demux13/5 -> Mux33/3  "C, Impurities, RE-2"
  Demux13/6 -> Mux33/4  "C, EcoRI enzyme, RE-2"
  Demux13/9 -> Mux36/3, Mux37/3  "C, Impurities, PE"
  Demux13/10 -> Mux36/4  "C, ECoRI Enzyme, PE"
  Mux36/1 -> "UF-101, C, R/P1"/2, "C, PE, 22"/1
  Demux15/3 -> Scope47/1
  Demux15/1 -> Scope45/1
  Demux15/10 -> Scope41/1
  Demux15/4 -> Scope38/1  "C, Impurities"
  AEX-301:304/1 -> "Output, AEX-301:304"/1, Demux15/1
  Demux15/12 -> Scope52/1
  Mux37/1 -> AEX-301:304/1, "Input, AEX-301:304"/1
  Demux15/16 -> Scope50/1
  Demux15/9 -> Scope42/1
  Demux15/8 -> Scope53/1  "C, pDNA"
  Demux15/6 -> Scope48/1
  Demux15/14 -> Scope37/1
  Demux15/11 -> Scope40/1
  Demux15/2 -> Scope46/1
  Demux15/7 -> Scope43/1
  Demux15/5 -> Scope35/1
  Demux15/15 -> Scope36/1
  Demux15/17 -> Scope49/1
  Demux15/13 -> Scope39/1
  Mux39/1 -> T-302/1
  T-302/1 -> Demux16/1
  Demux17/5 -> Mux41/4  "C, linpDNA"
  Demux17/3 -> Mux41/2  "C, Impurities"
  Demux17/6 -> Mux41/5  "C, Cleancap"
  Demux16/1 -> Subtract7/2, Mux40/1, Mux38/1  "Q"
  Demux16/2 -> "R-401, C IN/OUT1"/1, Mux40/3, Mux38/2  "C, linpDNA"
  R-401/1 -> Demux17/1
  Demux17/1 -> Subtract8/2, Scope55/1  "Volume"
  Demux17/2 -> Mux41/1  "C, mRNA"
  Mux40/1 -> R-401/1
  Demux17/4 -> Mux41/3  "C, T7 Enzyme"
  Demux17/8 -> Mux41/7  "C, Nucleotides"
  R-402/1 -> Demux18/1
  Demux18/2 -> Mux43/1  "C, mRNA"
  Demux18/3 -> Mux43/2  "C, Impurities"
  Demux18/4 -> Mux43/3  "C, T7 Enzyme"
  Demux18/5 -> Mux43/4  "C, linpDNA"
  Demux18/6 -> Mux43/5  "C, Cleancap"
  Demux18/8 -> Mux43/7  "C, Nucleotides"
  Demux18/9 -> Mux43/8  "C, Degraded products"
  Mux44/1 -> VSP-401/1(u)
  VSP-401/1(y) -> Demux20/1
  Mux45/1 -> Mux47/2
  UF-401/1(y) -> Demux19/1
  Demux19/4 -> Mux50/2, Mux46/2  "C, Impurities, RE"
  Demux19/5 -> Mux50/3, Mux46/3  "C, T7 Enzyme, RE"
  Demux19/6 -> Mux46/4  "C, linpDNA, RE"
  Demux19/7 -> Mux46/5  "C, CleanCap, RE"
  Demux19/9 -> Mux46/7  "C, Nucleotides, RE"
  Demux19/10 -> Mux46/8  "C, Degraded products, RE"
  Demux18/10 -> Mux43/9  "C, DNase I"
  Demux12/6 -> Scope63/1  "Level"
  Mux26/1 -> R-301/1
  Mux29/1 -> Scope6/1
  Mux34/1 -> "C, output"/1, Mux35/1
  Demux12/1 -> Subtract5/2, Scope12/1  "Volume"
  Mux46/1 -> "C, RE, 32"/1
  Mux48/1 -> "C, PE-2"/1
  Demux19/1 -> Scope60/1  "Q, PE-2"
  Mux42/1 -> R-402/1
  Demux18/11 -> Scope84/1  "Level"
  Demux23/3 -> Mux51/2, Mux49/3  "C, Impurities"
  Demux21/15 -> Scope66/1
  Demux21/1 -> Scope75/1
  Demux21/3 -> Scope77/1
  Demux21/10 -> Scope71/1
  Demux21/2 -> Scope76/1
  Demux21/6 -> Scope78/1
  Demux21/11 -> Scope70/1
  Demux21/17 -> Scope79/1
  Demux21/8 -> Mux55/4, Scope82/1  "C, impurities"
  Demux21/5 -> Scope58/1
  AC-401:404/1 -> "Output, AC-401:404"/1, Demux21/1
  Demux21/14 -> Scope67/1
  Demux21/16 -> Scope80/1
  Demux21/4 -> Scope68/1  "C, T7 enzyme"
  Demux21/9 -> Scope72/1
  Demux21/7 -> Scope73/1
  Demux21/13 -> Scope69/1
  Demux22/3 -> Scope87/1
  Demux22/10 -> Scope92/1
  Demux22/4 -> Scope101/1
  Demux22/6 -> Scope90/1  "C, Impurities"
  HIC-401:404/1 -> Demux22/1, "Output, HIC-401:404"/1
  Demux22/9 -> Scope93/1
  Demux22/7 -> Scope88/1
  Demux22/11 -> Scope91/1
  Mux51/1 -> "Intput, HIC-401:404"/1, HIC-401:404/1
  Mux50/1 -> AC-401:404/1, "Input, AC-401:404"/1
  Demux9/1 -> Neutralization,flow IN/OUT1/2, Mux12/1, "Total flow, out"/1  "Q, out"
  Demux18/1 -> Subtract9/2, Scope65/1  "Volume"
  Demux17/7 -> Mux41/6  "C, MgAcetate"
  Demux17/9 -> Scope56/1  "Level"
  Demux18/7 -> Mux43/6  "C, MgAcetate"
  Demux19/8 -> Mux46/6  "C, MgAcetate, RE"
  Demux19/11 -> Mux46/9  "C, DNase I ,RE"
  Demux19/12 -> Mux48/1  "C, mRNA, PE-2"
  Demux19/13 -> Mux48/2  "C, Impurities, PE-2"
  Demux19/14 -> Mux48/3  "C, T7 enzyme, PE-2"
  Demux19/15 -> Mux48/4  "C, linpDNA, PE-2"
  Demux19/16 -> Mux48/5  "C, CleanCap, PE-2"
  Demux19/17 -> Mux48/6  "C, MgAcetate, PE-2"
  Demux19/18 -> Mux48/7  "C, Nucleotides, PE-2"
  Demux19/19 -> Mux48/8  "C, Degraded products, PE-2"
  Demux19/20 -> Mux48/9  "C, DNase I, PE-2"
  Mux55/1 -> T-402/1
  T-402/1 -> Demux23/1
  Mux62/1 -> Mux63/2
  Demux25/2 -> Mux57/4  "C, solution"
  Mux64/1 -> Mux63/1, Scope51/1
  Demux28/3 -> Mux78/1, Mux58/1  "C, mRNA-LNP, RE"
  Mux61/1 -> VSP-503/1(u)
  Mux63/1 -> NF-501/1(u)
  T-501/1 -> Demux24/1
  Demux24/1 -> Subtract12/2, Mux91/1, Mux57/1  "Q, TankF"
  MM-501/1(y) -> Demux26/1
  Mux57/1 -> MM-501/1(u)
  Mux58/1 -> "C,RE, 47"/1
  Demux28/4 -> Mux58/2  "C, LNP, RE"
  Demux25/1 -> Mux57/3, Scope121/1, Subtract13/2  "Q, TankG"
  Demux28/2 -> Scope112/1, Mux74/1  "Q, RE-3"
  Demux24/2 -> Mux91/2, Mux57/2  "C, mRNA"
  Mux56/1 -> T-501/1
  VSP-503/1(y) -> Demux27/1
  M-501/1 -> Demux25/1
  Demux28/6 -> Mux78/2, Mux58/4  "C, Sucroce, RE"
  Demux28/5 -> Mux58/3  "C, Ethanol, RE"
  NF-501/1(y) -> Demux28/1
  Demux28/1 -> Scope111/1  "Q, PE, 47"
  Mux60/1 -> "C, PE-3"/1
  Mux72/1 -> "C, RE-3"/1
  VSP-504/1(y) -> Demux31/1
  Mux73/1 -> "C, mRNA-LNP, PE, 48"/1
  Demux32/2 -> Scope3/1  "Q, RE-3"
  Demux31/2 -> Subtract15/2, Scope124/1, Scope98/1, Mux80/2, Mux75/2  "P"
  MF-501/1(y) -> Demux32/1
  Demux32/1 -> Scope127/1  "Q, PE, 48"
  Demux32/3 -> Mux72/1  "C, mRNA-LNP, RE-3"
  Mux74/1 -> VSP-504/1(u)
  Mux75/1 -> Mux76/2
  Mux76/1 -> MF-501/1(u)
  Demux32/4 -> Mux72/2  "C, Sucrose, RE-3"
  Mux78/1 -> Mux76/1
  MATLAB Function1/1(y) -> Demux29/1
  Mux3/1 -> MATLAB Function1/1(u)
  Mux70/1 -> M-501/1
  Demux29/1 -> Scope16/1, Mux66/1  "Q, total"
  Demux29/2 -> Mux66/2  "C, LNP"
  Demux29/3 -> Mux66/3  "C, Ethanol"
  Demux29/4 -> Mux66/4  "C, sucrose"
  Demux29/5 -> Mux66/5  "C, Impurity 1"
  Mux66/1 -> Scope57/1, Mux70/1
  Demux26/2 -> Mux64/2  "C, LNP"
  Demux26/3 -> Mux64/3  "C, Ethanol"
  Demux26/4 -> Mux64/4  "C, Sucrose 1"
  MATLAB Function3/1(y) -> "Area, UF-301"/1, Mux35/3
  Mux67/1 -> MATLAB Function3/1(u)
  Mux69/1 -> MATLAB Function6/1(u)
  MATLAB Function6/1(y) -> "Area, UF-201"/1, Mux19/3
  Demux7/1 -> Mux69/1, Mux15/1  "Q"
  Demux7/2 -> Mux15/2, Scope107/1, Subtract3/2, Mux69/2  "P"
  Mux68/1 -> MATLAB Function14/1(u)
  MATLAB Function14/1(y) -> Mux47/3
  Demux20/1 -> Scope31/1, Mux68/1, Mux45/1  "Q"
  Demux20/2 -> Mux45/2, Mux68/2, Subtract10/2, Scope32/1  "P"
  Mux59/1 -> MATLAB Function15/1(u)
  MATLAB Function15/1(y) -> Mux63/3
  Demux27/1 -> Mux59/1, Mux62/1  "Q"
  Demux27/2 -> Mux59/2, Mux62/2, Scope123/1, Subtract14/2  "P"
  MATLAB Function18/1(y) -> Mux76/3
  Demux31/1 -> Mux80/1, Mux75/1  "Q"
  Mux80/1 -> MATLAB Function18/1(u)
  Demux22/5 -> Scope100/1
  Demux22/2 -> Scope85/1
  Demux22/1 -> Scope89/1
  Demux29/6 -> Mux66/6  "C, Impurity 2"
  Demux26/5 -> Mux64/5  "C, Impurity 1"
  Demux28/7 -> Mux58/5  "C, Impurity 1, RE"
  Demux32/5 -> Mux72/3  "C, Impurity 2, RE-3"
  Demux32/6 -> Mux73/1  "C, mRNA-LNP, PE"
  Demux32/7 -> Mux73/2  "C, Sucrose, PE"
  Demux32/8 -> Mux73/3  "C, Impurity 2, PE"
  Demux/4 -> Mux25/3, Mux1/3  "C, N"
  Demux/3 -> Mux1/2, Mux25/2  "C, Glu"
  Demux/2 -> Mux25/1, Mux1/1  "C, X"
  Mux47/1 -> Scope27/1, UF-401/1(u)
  Mux38/1 -> Scope54/1
  Demux26/1 -> Mux64/1  "C, mRNA-LNP"
  Demux/1 -> "R-101, Volume+height"/1, Subtract/2, "R-101, Volume"/1  "V"
  Mux49/1 -> Scope4/1
  Mux13/1 -> "UF-101, C, R/P"/1, "C, RE, 4"/1
  Demux3/2 -> Subtract1/2, "Pressure, P"/1, Mux6/2  "P"
  Mux71/1 -> "R-101, C:IN,OUT"/1
  Mux25/1 -> "R-101, C:IN,OUT"/2
  Mux10/1 -> "UF-101, C, R/P"/2, Mux/4, "C, PE-1"/1
  Mux79/1 -> "Tank-101, IN/OUT"/1
  Mux81/1 -> "R-201, C,byproduct"/1
  Mux82/1 -> "R-201, C,byproduct"/2
  Mux83/1 -> "R-201, C,x"/2
  Demux6/2 -> "UF-201, Q, R/P2"/1, "Q, RE-1"/1  "Q, RE. 4"
  Mux84/1 -> AEX:201:204 C/2
  Mux85/1 -> AEX:201:204 C/1
  T-205/1 -> "Tank-205, IN/OUT1"/2, Demux11/1
  Mux86/1 -> "Tank-205, IN/OUT1"/1
  Demux6/1 -> Mux20/2, "UF-201, Q, R/P2"/2, AEX:201:204,Q IN/OUT1/1, Mux27/1, AEX:201:204,Q IN/OUT1/2, Mux86/1, "Q, PE, 14"/1  "Q, RE. 4"
  Demux10/18 -> Mux86/2, Mux30/2, Scope/1, Mux84/1, Mux20/3  "C, pDNA,  RE"
  Mux88/1 -> "R-301, C IN/OUT2"/2
  Mux41/1 -> "R-401, C IN/OUT1"/2, IVT/1, "R-402, C IN/OUT2"/1, Mux42/3
  Mux43/1 -> "R-402, C IN/OUT2"/2, Scope9/1, Mux47/1
  Demux21/18 -> Scope14/1  "C, mRNA"
  Demux22/12 -> Scope15/1  "C, mRNA"
  Mux20/1 -> Scope62/1, MATLAB Function/1(u)
  Demux13/8 -> Mux36/2, Mux87/1, Mux37/4  "C, linpDNA, PE"
  Demux13/1 -> "UF-101, Q, R/P1"/2, Scope33/1, Mux87/2, Scope11/1, Mux37/1  "Q, RE. 4"
  Demux13/7 -> Mux36/1, Mux37/2  "C, pDNA, PE"
  Mux87/1 -> Scope74/1, MATLAB Function2/1(u)
  Demux15/18 -> Mux87/3, Scope10/1, Mux39/2  "C, pDNA,  RE"
  MATLAB Function2/1(y) -> Mux39/1, Scope64/1
  Demux19/3 -> Mux89/1, Mux50/4, Mux46/1  "C, mRNA, PE"
  Demux19/2 -> Scope1/1, Mux89/2, Mux50/1  "Q, RE. 4"
  MATLAB Function7/1(y) -> Mux55/1, Scope83/1
  Mux89/1 -> Scope86/1, MATLAB Function7/1(u)
  Demux21/12 -> Mux89/3, Mux55/2, Scope81/1  "C, mRNA,  RE"
  Mux90/1 -> Scope95/1, MATLAB Function10/1(u)
  Demux23/1 -> Subtract11/2, Mux90/2, Mux49/1, Mux51/1  "Q, RE. 4"
  Demux23/2 -> Mux51/3, Mux90/1, Mux49/2  "C, mRNA, PE"
  Demux22/8 -> Mux90/3, Mux56/2, Mux3/2, Scope103/1  "C, mRNA,  RE"
  MATLAB Function10/1(y) -> Mux3/1, Mux56/1, Scope94/1
  MATLAB Function/1(y) -> Mux30/1, Scope61/1
  Mux91/1 -> Scope59/1
  Demux26/6 -> Mux64/6  "C, Impurity 2"
  Demux26/7 -> Scope96/1, Mux61/1  "Q, total"
  Demux28/8 -> Mux78/3, Mux58/6  "C,imurity 2 PE-3"
  Demux28/9 -> Mux60/1  "C, mRNA-LNP, PE-3"
  Demux28/10 -> Mux60/2  "C, LNP, PE-3"
  Demux28/11 -> Mux60/3  "C, Ethanol, PE-3"
  Demux28/12 -> Mux60/4  "C, Sucrose, PE-3"
  Demux28/13 -> Mux60/5  "C, Impurity 1, PE-3"
  Demux28/14 -> Mux60/6  "C, Impurity 2, PE-3"
  Constant/1 -> Subtract/1
  Subtract/1 -> PID Controller/1
  PID Controller/1 -> Mux4/1, Scope102/1, Mux2/5
  Constant1/1 -> Subtract1/1
  Subtract1/1 -> PID Controller1/1
  PID Controller1/1 -> Scope104/1, Mux4/2
  Constant2/1 -> Subtract2/1
  Subtract2/1 -> PID Controller2/1
  PID Controller2/1 -> Scope105/1, Mux9/3
  Subtract3/1 -> PID Controller3/1
  Constant3/1 -> Subtract3/1
  PID Controller3/1 -> Scope106/1, Mux12/2
  Constant4/1 -> Subtract4/1
  Subtract4/1 -> PID Controller4/1
  PID Controller4/1 -> Scope108/1, Mux30/3
  Constant5/1 -> Subtract5/1
  Subtract5/1 -> PID Controller5/1
  PID Controller5/1 -> Scope109/1, Mux31/1, Mux26/2
  Constant6/1 -> Subtract6/1
  Subtract6/1 -> PID Controller6/1
  PID Controller6/1 -> Scope113/1, Mux31/2
  Constant7/1 -> Subtract7/1
  Subtract7/1 -> PID Controller7/1
  PID Controller7/1 -> Mux39/3, Scope114/1
  Constant8/1 -> Subtract8/1
  Subtract8/1 -> PID Controller8/1
  PID Controller8/1 -> Scope17/1, Mux42/1, Mux40/2, Scope115/1
  Constant9/1 -> Subtract9/1
  Subtract9/1 -> PID Controller9/1
  PID Controller9/1 -> Scope116/1, Mux42/2, Mux44/1
  Constant10/1 -> Subtract10/1
  Subtract10/1 -> PID Controller10/1
  PID Controller10/1 -> Scope117/1, Mux44/2
  Constant11/1 -> Subtract11/1
  Subtract11/1 -> PID Controller11/1
  PID Controller11/1 -> Scope118/1, Mux55/3
  Constant13/1 -> Subtract13/1
  Subtract13/1 -> PID Controller13/1
  PID Controller13/1 -> Mux70/2, Scope120/1
  Constant12/1 -> Subtract12/1
  Subtract12/1 -> PID Controller12/1
  PID Controller12/1 -> Scope119/1, Mux56/3
  PID Controller14/1 -> Mux61/2, Scope122/1
  Subtract14/1 -> PID Controller14/1
  Constant14/1 -> Subtract14/1
  Constant15/1 -> Subtract15/1
  Subtract15/1 -> PID Controller15/1
  PID Controller15/1 -> Scope125/1, Mux74/2
  MATLAB Function8/1(y) -> Mux8/1, Mux/2
  Clock/1 -> MATLAB Function8/2(t)
  Constant16/1 -> Mux8/2, MATLAB Function8/1(value)
  "C, Glu, media [g/L]"/1 -> Mux14/2
  "C, N, media [g/L]"/1 -> Mux14/3
  Mux14/1 -> Mux/3
  "C, X, media [g/L]"/1 -> Mux14/1
  Mux8/1 -> Scope128/1
